simulink model "ieee30"  (R2017a)
settings: Solver=VariableStepDiscrete  StartTime=0.0  StopTime=0.012  MaxStep=1e-4  RelTol=1e-3
undefined symbols (not defined in the file): Angle, Magnitude
libraries: powerlib x548
(part 1 of 4)
settings Model: Creator=wynston  LastModifiedBy=Wynston
settings DataIOCC: ReturnWorkspaceOutputsName=simout

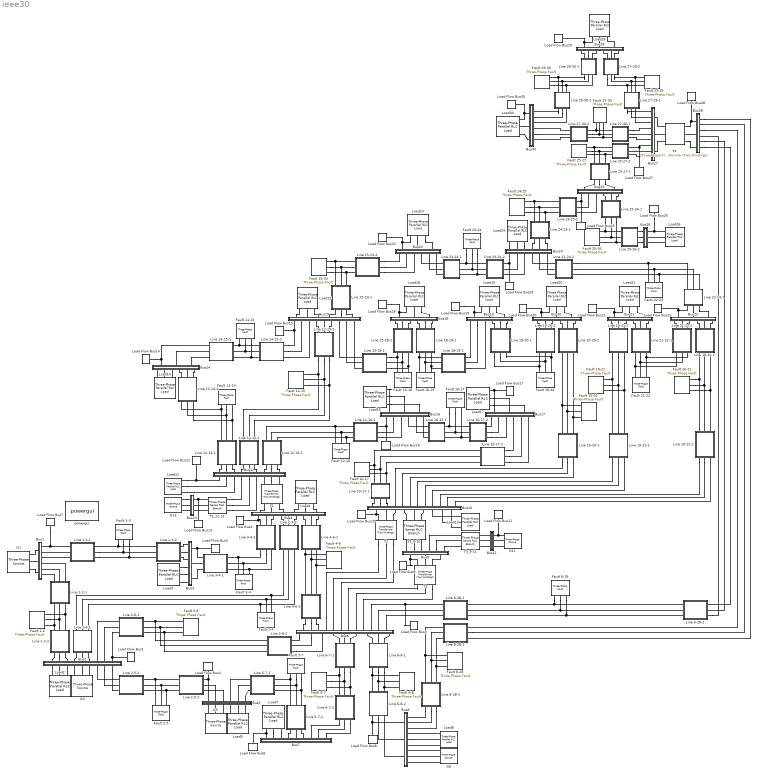
== system ieee30 ==
  Bus1 : Subsystem
  Bus10 : Subsystem
  Bus11 : Subsystem
  Bus12 : Subsystem
  Bus13 : Subsystem
  Bus14 : Subsystem
  Bus15 : Subsystem
  Bus16 : Subsystem
  Bus17 : Subsystem
  Bus18 : Subsystem
  Bus19 : Subsystem
  Bus2 : Subsystem
  Bus20 : Subsystem
  Bus21 : Subsystem
  Bus22 : Subsystem
  Bus23 : Subsystem
  Bus24 : Subsystem
  Bus25 : Subsystem
  Bus26 : Subsystem
  Bus27 : Subsystem
  Bus28 : Subsystem
  Bus29 : Subsystem
  Bus3 : Subsystem
  Bus30 : Subsystem
  Bus4 : Subsystem
  Bus5 : Subsystem
  Bus6 : Subsystem
  Bus7 : Subsystem
  Bus8 : Subsystem
  Bus9 : Subsystem
  Fault 1-2 : powerlib/Elements/Three-Phase Fault  InitialStates=0  FaultA=off  FaultB=off  FaultC=off  GroundFault=off  SwitchTimes=[0.008 0.1]  External=off  SwitchStatus=NaN  FaultResistance=0.001  GroundResistance=0.001  SnubberResistance=1e6  SnubberCapacitance=inf  Measurements=None
  Fault 1-3 : powerlib/Elements/Three-Phase Fault  InitialStates=0  FaultA=off  FaultB=off  FaultC=off  GroundFault=off  SwitchTimes=[0.008 0.1]  External=off  SwitchStatus=NaN  FaultResistance=0.001  GroundResistance=0.001  SnubberResistance=1e6  SnubberCapacitance=inf  Measurements=None
  Fault 10-{17,20..22} (4 alike) : powerlib/Elements/Three-Phase Fault  InitialStates=0  FaultA=off  FaultB=off  FaultC=off  GroundFault=off  SwitchTimes=[0.008 0.1]  External=off  SwitchStatus=NaN  FaultResistance=0.001  GroundResistance=0.001  SnubberResistance=1e6  SnubberCapacitance=inf  Measurements=None
  Fault 12-14 : powerlib/Elements/Three-Phase Fault  InitialStates=0  FaultA=off  FaultB=off  FaultC=off  GroundFault=off  SwitchTimes=[0.008 0.1]  External=off  SwitchStatus=NaN  FaultResistance=0.001  GroundResistance=0.001  SnubberResistance=1e6  SnubberCapacitance=inf  Measurements=None
  Fault 12-15 : powerlib/Elements/Three-Phase Fault  InitialStates=0  FaultA=off  FaultB=off  FaultC=off  GroundFault=off  SwitchTimes=[0.008 0.1]  External=off  SwitchStatus=NaN  FaultResistance=0.001  GroundResistance=0.001  SnubberResistance=1e6  SnubberCapacitance=inf  Measurements=None
  Fault 12-16 : powerlib/Elements/Three-Phase Fault  InitialStates=0  FaultA=off  FaultB=off  FaultC=off  GroundFault=off  SwitchTimes=[0.008 0.1]  External=off  SwitchStatus=NaN  FaultResistance=0.001  GroundResistance=0.001  SnubberResistance=1e6  SnubberCapacitance=inf  Measurements=None
  Fault 14-15 : powerlib/Elements/Three-Phase Fault  InitialStates=0  FaultA=off  FaultB=off  FaultC=off  GroundFault=off  SwitchTimes=[0.008 0.1]  External=off  SwitchStatus=NaN  FaultResistance=0.001  GroundResistance=0.001  SnubberResistance=1e6  SnubberCapacitance=inf  Measurements=None
  Fault 15-18 : powerlib/Elements/Three-Phase Fault  InitialStates=0  FaultA=off  FaultB=off  FaultC=off  GroundFault=off  SwitchTimes=[0.008 0.1]  External=off  SwitchStatus=NaN  FaultResistance=0.001  GroundResistance=0.001  SnubberResistance=1e6  SnubberCapacitance=inf  Measurements=None
  Fault 15-23 : powerlib/Elements/Three-Phase Fault  InitialStates=0  FaultA=off  FaultB=off  FaultC=off  GroundFault=off  SwitchTimes=[0.008 0.1]  External=off  SwitchStatus=NaN  FaultResistance=0.001  GroundResistance=0.001  SnubberResistance=1e6  SnubberCapacitance=inf  Measurements=None
  Fault 16-17 : powerlib/Elements/Three-Phase Fault  InitialStates=0  FaultA=off  FaultB=off  FaultC=off  GroundFault=off  SwitchTimes=[0.008 0.1]  External=off  SwitchStatus=NaN  FaultResistance=0.001  GroundResistance=0.001  SnubberResistance=1e6  SnubberCapacitance=inf  Measurements=None
  Fault 18-19 : powerlib/Elements/Three-Phase Fault  InitialStates=0  FaultA=off  FaultB=off  FaultC=off  GroundFault=off  SwitchTimes=[0.008 0.1]  External=off  SwitchStatus=NaN  FaultResistance=0.001  GroundResistance=0.001  SnubberResistance=1e6  SnubberCapacitance=inf  Measurements=None
  Fault 19-20 : powerlib/Elements/Three-Phase Fault  InitialStates=0  FaultA=off  FaultB=off  FaultC=off  GroundFault=off  SwitchTimes=[0.008 0.1]  External=off  SwitchStatus=NaN  FaultResistance=0.001  GroundResistance=0.001  SnubberResistance=1e6  SnubberCapacitance=inf  Measurements=None
  Fault 2-4 : powerlib/Elements/Three-Phase Fault  InitialStates=0  FaultA=off  FaultB=off  FaultC=off  GroundFault=off  SwitchTimes=[0.008 0.1]  External=off  SwitchStatus=NaN  FaultResistance=0.001  GroundResistance=0.001  SnubberResistance=1e6  SnubberCapacitance=inf  Measurements=None
  Fault 2-5 : powerlib/Elements/Three-Phase Fault  InitialStates=0  FaultA=off  FaultB=off  FaultC=off  GroundFault=off  SwitchTimes=[0.008 0.1]  External=off  SwitchStatus=NaN  FaultResistance=0.001  GroundResistance=0.001  SnubberResistance=1e6  SnubberCapacitance=inf  Measurements=None
  Fault 2-6 : powerlib/Elements/Three-Phase Fault  InitialStates=0  FaultA=off  FaultB=off  FaultC=off  GroundFault=off  SwitchTimes=[0.008 0.1]  External=off  SwitchStatus=NaN  FaultResistance=0.001  GroundResistance=0.001  SnubberResistance=1e6  SnubberCapacitance=inf  Measurements=None
  Fault 21-22 : powerlib/Elements/Three-Phase Fault  InitialStates=0  FaultA=off  FaultB=off  FaultC=off  GroundFault=off  SwitchTimes=[0.008 0.1]  External=off  SwitchStatus=NaN  FaultResistance=0.001  GroundResistance=0.001  SnubberResistance=1e6  SnubberCapacitance=inf  Measurements=None
  Fault 22-24 : powerlib/Elements/Three-Phase Fault  InitialStates=0  FaultA=off  FaultB=off  FaultC=off  GroundFault=off  SwitchTimes=[0.008 0.1]  External=off  SwitchStatus=NaN  FaultResistance=0.001  GroundResistance=0.001  SnubberResistance=1e6  SnubberCapacitance=inf  Measurements=None
  Fault 23-24 : powerlib/Elements/Three-Phase Fault  InitialStates=0  FaultA=off  FaultB=off  FaultC=off  GroundFault=off  SwitchTimes=[0.008 0.1]  External=off  SwitchStatus=NaN  FaultResistance=0.001  GroundResistance=0.001  SnubberResistance=1e6  SnubberCapacitance=inf  Measurements=None
  Fault 24-25 : powerlib/Elements/Three-Phase Fault  InitialStates=0  FaultA=off  FaultB=off  FaultC=off  GroundFault=off  SwitchTimes=[0.008 0.1]  External=off  SwitchStatus=NaN  FaultResistance=0.001  GroundResistance=0.001  SnubberResistance=1e6  SnubberCapacitance=inf  Measurements=None
  Fault 25-26 : powerlib/Elements/Three-Phase Fault  InitialStates=0  FaultA=off  FaultB=off  FaultC=off  GroundFault=off  SwitchTimes=[0.008 0.1]  External=off  SwitchStatus=NaN  FaultResistance=0.001  GroundResistance=0.001  SnubberResistance=1e6  SnubberCapacitance=inf  Measurements=None
  Fault 25-27 : powerlib/Elements/Three-Phase Fault  InitialStates=0  FaultA=off  FaultB=off  FaultC=off  GroundFault=off  SwitchTimes=[0.008 0.1]  External=off  SwitchStatus=NaN  FaultResistance=0.001  GroundResistance=0.001  SnubberResistance=1e6  SnubberCapacitance=inf  Measurements=None
  Fault 27-29 : powerlib/Elements/Three-Phase Fault  InitialStates=0  FaultA=off  FaultB=off  FaultC=off  GroundFault=off  SwitchTimes=[0.008 0.1]  External=off  SwitchStatus=NaN  FaultResistance=0.001  GroundResistance=0.001  SnubberResistance=1e6  SnubberCapacitance=inf  Measurements=None
  Fault 27-30 : powerlib/Elements/Three-Phase Fault  InitialStates=0  FaultA=off  FaultB=off  FaultC=off  GroundFault=off  SwitchTimes=[0.008 0.1]  External=off  SwitchStatus=NaN  FaultResistance=0.001  GroundResistance=0.001  SnubberResistance=1e6  SnubberCapacitance=inf  Measurements=None
  Fault 29-30 : powerlib/Elements/Three-Phase Fault  InitialStates=0  FaultA=off  FaultB=off  FaultC=off  GroundFault=off  SwitchTimes=[0.008 0.1]  External=off  SwitchStatus=NaN  FaultResistance=0.001  GroundResistance=0.001  SnubberResistance=1e6  SnubberCapacitance=inf  Measurements=None
  Fault 3-4 : powerlib/Elements/Three-Phase Fault  InitialStates=0  FaultA=off  FaultB=off  FaultC=off  GroundFault=off  SwitchTimes=[0.008 0.1]  External=off  SwitchStatus=NaN  FaultResistance=0.001  GroundResistance=0.001  SnubberResistance=1e6  SnubberCapacitance=inf  Measurements=None
  Fault 4-6 : powerlib/Elements/Three-Phase Fault  InitialStates=0  FaultA=off  FaultB=off  FaultC=off  GroundFault=off  SwitchTimes=[0.008 0.1]  External=off  SwitchStatus=NaN  FaultResistance=0.001  GroundResistance=0.001  SnubberResistance=1e6  SnubberCapacitance=inf  Measurements=None
  Fault 5-7 : powerlib/Elements/Three-Phase Fault  InitialStates=0  FaultA=off  FaultB=off  FaultC=off  GroundFault=off  SwitchTimes=[0.008 0.1]  External=off  SwitchStatus=NaN  FaultResistance=0.001  GroundResistance=0.001  SnubberResistance=1e6  SnubberCapacitance=inf  Measurements=None
  Fault 6-28 : powerlib/Elements/Three-Phase Fault  InitialStates=0  FaultA=off  FaultB=off  FaultC=off  GroundFault=off  SwitchTimes=[0.008 0.1]  External=off  SwitchStatus=NaN  FaultResistance=0.001  GroundResistance=0.001  SnubberResistance=1e6  SnubberCapacitance=inf  Measurements=None
  Fault 6-7 : powerlib/Elements/Three-Phase Fault  InitialStates=0  FaultA=off  FaultB=off  FaultC=off  GroundFault=off  SwitchTimes=[0.008 0.1]  External=off  SwitchStatus=NaN  FaultResistance=0.001  GroundResistance=0.001  SnubberResistance=1e6  SnubberCapacitance=inf  Measurements=None
  Fault 6-8 : powerlib/Elements/Three-Phase Fault  InitialStates=0  FaultA=off  FaultB=off  FaultC=off  GroundFault=off  SwitchTimes=[0.008 0.1]  External=off  SwitchStatus=NaN  FaultResistance=0.001  GroundResistance=0.001  SnubberResistance=1e6  SnubberCapacitance=inf  Measurements=None
  Fault 8-28 : powerlib/Elements/Three-Phase Fault  InitialStates=0  FaultA=off  FaultB=off  FaultC=off  GroundFault=off  SwitchTimes=[0.008 0.1]  External=off  SwitchStatus=NaN  FaultResistance=0.001  GroundResistance=0.001  SnubberResistance=1e6  SnubberCapacitance=inf  Measurements=None
  G1 : powerlib/Electrical Sources/Three-Phase Source  InternalConnection=Yg  VoltagePhases=off  Voltage=(132000)*2.93771  PhaseAngle=58.3306  Voltage_phases=[25e3 25e3 25e3]/sqrt(3)  PhaseAngles_phases=[0 -120 +120]  Frequency=60  NonIdealSource=on  SpecifyImpedance=on  Resistance=0.8929  Inductance=16.58e-3  ShortCircuitLevel=100e6  BaseVoltage=132e3  XRratio=100000  BusType=swing  Pref=0e6  Qref=0  Prefabc=[10e3, 10e3, 10e3]  Qrefabc=[0, 0, 0]  Qmin=0e6  Qmax=0e6
  G11 : powerlib/Electrical Sources/Three-Phase Source  InternalConnection=Yg  VoltagePhases=off  Voltage=(33000)*1.10022  PhaseAngle=-11.1711  Voltage_phases=[25e3 25e3 25e3]/sqrt(3)  PhaseAngles_phases=[0 -120 +120]  Frequency=60  NonIdealSource=on  SpecifyImpedance=on  Resistance=0.8929  Inductance=16.58e-3  ShortCircuitLevel=100e6  BaseVoltage=33e3  XRratio=100000  BusType=PV  Pref=0e6  Qref=0  Prefabc=[10e3, 10e3, 10e3]  Qrefabc=[0, 0, 0]  Qmin=-6e6  Qmax=24e6
  G13 : powerlib/Electrical Sources/Three-Phase Source  InternalConnection=Yg  VoltagePhases=off  Voltage=(33000)*1.10798  PhaseAngle=-18.3402  Voltage_phases=[25e3 25e3 25e3]/sqrt(3)  PhaseAngles_phases=[0 -120 +120]  Frequency=60  NonIdealSource=on  SpecifyImpedance=on  Resistance=0.8929  Inductance=16.58e-3  ShortCircuitLevel=100e6  BaseVoltage=32e3  XRratio=100000  BusType=PV  Pref=0e6  Qref=0  Prefabc=[10e3, 10e3, 10e3]  Qrefabc=[0, 0, 0]  Qmin=-6e6  Qmax=24e6
  G2 : powerlib/Electrical Sources/Three-Phase Source  InternalConnection=Yg  VoltagePhases=off  Voltage=(132000)*1.55993  PhaseAngle=9.4414  Voltage_phases=[25e3 25e3 25e3]/sqrt(3)  PhaseAngles_phases=[0 -120 +120]  Frequency=60  NonIdealSource=on  SpecifyImpedance=on  Resistance=0.8929  Inductance=16.58e-3  ShortCircuitLevel=100e6  BaseVoltage=132e3  XRratio=100000  BusType=PV  Pref=40e6  Qref=0  Prefabc=[10e3, 10e3, 10e3]  Qrefabc=[0, 0, 0]  Qmin=-40e6  Qmax=50e6
  G5 : powerlib/Electrical Sources/Three-Phase Source  InternalConnection=Yg  VoltagePhases=off  Voltage=(132000)*1.38256  PhaseAngle=-14.4167  Voltage_phases=[25e3 25e3 25e3]/sqrt(3)  PhaseAngles_phases=[0 -120 +120]  Frequency=60  NonIdealSource=on  SpecifyImpedance=on  Resistance=0.8929  Inductance=16.58e-3  ShortCircuitLevel=100e6  BaseVoltage=132e3  XRratio=100000  BusType=PV  Pref=0e6  Qref=0  Prefabc=[10e3, 10e3, 10e3]  Qrefabc=[0, 0, 0]  Qmin=-40e6  Qmax=40e6
  G8 : powerlib/Electrical Sources/Three-Phase Source  InternalConnection=Yg  VoltagePhases=off  Voltage=(132000)*1.37308  PhaseAngle=-11.5895  Voltage_phases=[25e3 25e3 25e3]/sqrt(3)  PhaseAngles_phases=[0 -120 +120]  Frequency=60  NonIdealSource=on  SpecifyImpedance=on  Resistance=0.8929  Inductance=16.58e-3  ShortCircuitLevel=100e6  BaseVoltage=132e3  XRratio=100000  BusType=PV  Pref=0e6  Qref=0  Prefabc=[10e3, 10e3, 10e3]  Qrefabc=[0, 0, 0]  Qmin=-10e6  Qmax=40e6
  Line 1-2-1 : Subsystem  mask{R=0.0096, X=0.02875, B=0.0132, MVA=100, KV=132}
      mask prompts: R "Resistance (pu)"; X "Reactance(pu)"; B "Susceptance (pu)(B/2)"; MVA "MVA Base"; KV "KV Base"
      mask help: Transmission Line Pi model
      mask init:
      | rt = R*(KV^2)/MVA;
      | lt = (X/377)*(KV^2)/MVA;
      | ct = (2*B/377)/((KV^2)/MVA);
      | ro = 2.5*R*(KV^2)/MVA;
      | lo = 2.5*(X/377)*(KV^2)/MVA;
      | co = (2*B/377)/((1.6*KV^2)/MVA);
      mask Display:
      | plot([0.2 0.8 0.8 0.2 0.2], [0.35 0.35 0.65 0.65 0.35]);
      | text(0.5, 0.5, 'π', 'horizontalAlignment', 'center');
  Line 1-2-2 : Subsystem  mask{R=0.0096, X=0.02875, B=0.0132, MVA=100, KV=132}
      mask prompts: R "Resistance (pu)"; X "Reactance(pu)"; B "Susceptance (pu)(B/2)"; MVA "MVA Base"; KV "KV Base"
      mask help: Transmission Line Pi model
      mask init:
      | rt = R*(KV^2)/MVA;
      | lt = (X/377)*(KV^2)/MVA;
      | ct = (2*B/377)/((KV^2)/MVA);
      | ro = 2.5*R*(KV^2)/MVA;
      | lo = 2.5*(X/377)*(KV^2)/MVA;
      | co = (2*B/377)/((1.6*KV^2)/MVA);
      mask Display:
      | plot([0.2 0.8 0.8 0.2 0.2], [0.35 0.35 0.65 0.65 0.35]);
      | text(0.5, 0.5, 'π', 'horizontalAlignment', 'center');
  Line 1-3-1 : Subsystem  mask{R=0.0226, X=0.0825, B=0.0102, MVA=100, KV=132}
      mask prompts: R "Resistance (pu)"; X "Reactance(pu)"; B "Susceptance (pu)(B/2)"; MVA "MVA Base"; KV "KV Base"
      mask help: Transmission Line Pi model
      mask init:
      | rt = R*(KV^2)/MVA;
      | lt = (X/377)*(KV^2)/MVA;
      | ct = (2*B/377)/((KV^2)/MVA);
      | ro = 2.5*R*(KV^2)/MVA;
      | lo = 2.5*(X/377)*(KV^2)/MVA;
      | co = (2*B/377)/((1.6*KV^2)/MVA);
      mask Display:
      | plot([0.2 0.8 0.8 0.2 0.2], [0.35 0.35 0.65 0.65 0.35]);
      | text(0.5, 0.5, 'π', 'horizontalAlignment', 'center');
  Line 1-3-2 : Subsystem  mask{R=0.0226, X=0.0825, B=0.0102, MVA=100, KV=132}
      mask prompts: R "Resistance (pu)"; X "Reactance(pu)"; B "Susceptance (pu)(B/2)"; MVA "MVA Base"; KV "KV Base"
      mask help: Transmission Line Pi model
      mask init:
      | rt = R*(KV^2)/MVA;
      | lt = (X/377)*(KV^2)/MVA;
      | ct = (2*B/377)/((KV^2)/MVA);
      | ro = 2.5*R*(KV^2)/MVA;
      | lo = 2.5*(X/377)*(KV^2)/MVA;
      | co = (2*B/377)/((1.6*KV^2)/MVA);
      mask Display:
      | plot([0.2 0.8 0.8 0.2 0.2], [0.35 0.35 0.65 0.65 0.35]);
      | text(0.5, 0.5, 'π', 'horizontalAlignment', 'center');
  Line 10-17-1 : Subsystem  mask{R=0.0162, X=0.04225, B=2.5e-05, MVA=100, KV=33}
      mask prompts: R "Resistance (pu)"; X "Reactance(pu)"; B "Susceptance (pu)(B/2)"; MVA "MVA Base"; KV "KV Base"
      mask help: Transmission Line Pi model
      mask init:
      | rt = R*(KV^2)/MVA;
      | lt = (X/377)*(KV^2)/MVA;
      | ct = (2*B/377)/((KV^2)/MVA);
      | ro = 2.5*R*(KV^2)/MVA;
      | lo = 2.5*(X/377)*(KV^2)/MVA;
      | co = (2*B/377)/((1.6*KV^2)/MVA);
      mask Display:
      | plot([0.2 0.8 0.8 0.2 0.2], [0.35 0.35 0.65 0.65 0.35]);
      | text(0.5, 0.5, 'π', 'horizontalAlignment', 'center');
  Line 10-17-2 : Subsystem  mask{R=0.0162, X=0.04225, B=2.5e-05, MVA=100, KV=33}
      mask prompts: R "Resistance (pu)"; X "Reactance(pu)"; B "Susceptance (pu)(B/2)"; MVA "MVA Base"; KV "KV Base"
      mask help: Transmission Line Pi model
      mask init:
      | rt = R*(KV^2)/MVA;
      | lt = (X/377)*(KV^2)/MVA;
      | ct = (2*B/377)/((KV^2)/MVA);
      | ro = 2.5*R*(KV^2)/MVA;
      | lo = 2.5*(X/377)*(KV^2)/MVA;
      | co = (2*B/377)/((1.6*KV^2)/MVA);
      mask Display:
      | plot([0.2 0.8 0.8 0.2 0.2], [0.35 0.35 0.65 0.65 0.35]);
      | text(0.5, 0.5, 'π', 'horizontalAlignment', 'center');
  Line 10-20-1 : Subsystem  mask{R=0.0468, X=0.1045, B=2.5e-05, MVA=100, KV=33}
      mask prompts: R "Resistance (pu)"; X "Reactance(pu)"; B "Susceptance (pu)(B/2)"; MVA "MVA Base"; KV "KV Base"
      mask help: Transmission Line Pi model
      mask init:
      | rt = R*(KV^2)/MVA;
      | lt = (X/377)*(KV^2)/MVA;
      | ct = (2*B/377)/((KV^2)/MVA);
      | ro = 2.5*R*(KV^2)/MVA;
      | lo = 2.5*(X/377)*(KV^2)/MVA;
      | co = (2*B/377)/((1.6*KV^2)/MVA);
      mask Display:
      | plot([0.2 0.8 0.8 0.2 0.2], [0.35 0.35 0.65 0.65 0.35]);
      | text(0.5, 0.5, 'π', 'horizontalAlignment', 'center');
  Line 10-20-2 : Subsystem  mask{R=0.0468, X=0.1045, B=2.5e-05, MVA=100, KV=33}
      mask prompts: R "Resistance (pu)"; X "Reactance(pu)"; B "Susceptance (pu)(B/2)"; MVA "MVA Base"; KV "KV Base"
      mask help: Transmission Line Pi model
      mask init:
      | rt = R*(KV^2)/MVA;
      | lt = (X/377)*(KV^2)/MVA;
      | ct = (2*B/377)/((KV^2)/MVA);
      | ro = 2.5*R*(KV^2)/MVA;
      | lo = 2.5*(X/377)*(KV^2)/MVA;
      | co = (2*B/377)/((1.6*KV^2)/MVA);
      mask Display:
      | plot([0.2 0.8 0.8 0.2 0.2], [0.35 0.35 0.65 0.65 0.35]);
      | text(0.5, 0.5, 'π', 'horizontalAlignment', 'center');
  Line 10-21-1 : Subsystem  mask{R=0.0174, X=0.03745, B=2.5e-05, MVA=100, KV=33}
      mask prompts: R "Resistance (pu)"; X "Reactance(pu)"; B "Susceptance (pu)(B/2)"; MVA "MVA Base"; KV "KV Base"
      mask help: Transmission Line Pi model
      mask init:
      | rt = R*(KV^2)/MVA;
      | lt = (X/377)*(KV^2)/MVA;
      | ct = (2*B/377)/((KV^2)/MVA);
      | ro = 2.5*R*(KV^2)/MVA;
      | lo = 2.5*(X/377)*(KV^2)/MVA;
      | co = (2*B/377)/((1.6*KV^2)/MVA);
      mask Display:
      | plot([0.2 0.8 0.8 0.2 0.2], [0.35 0.35 0.65 0.65 0.35]);
      | text(0.5, 0.5, 'π', 'horizontalAlignment', 'center');
  Line 10-21-2 : Subsystem  mask{R=0.0174, X=0.03745, B=2.5e-05, MVA=100, KV=33}
      mask prompts: R "Resistance (pu)"; X "Reactance(pu)"; B "Susceptance (pu)(B/2)"; MVA "MVA Base"; KV "KV Base"
      mask help: Transmission Line Pi model
      mask init:
      | rt = R*(KV^2)/MVA;
      | lt = (X/377)*(KV^2)/MVA;
      | ct = (2*B/377)/((KV^2)/MVA);
      | ro = 2.5*R*(KV^2)/MVA;
      | lo = 2.5*(X/377)*(KV^2)/MVA;
      | co = (2*B/377)/((1.6*KV^2)/MVA);
      mask Display:
      | plot([0.2 0.8 0.8 0.2 0.2], [0.35 0.35 0.65 0.65 0.35]);
      | text(0.5, 0.5, 'π', 'horizontalAlignment', 'center');
  Line 10-22-1 : Subsystem  mask{R=0.03635, X=0.075, B=2.5e-05, MVA=100, KV=33}
      mask prompts: R "Resistance (pu)"; X "Reactance(pu)"; B "Susceptance (pu)(B/2)"; MVA "MVA Base"; KV "KV Base"
      mask help: Transmission Line Pi model
      mask init:
      | rt = R*(KV^2)/MVA;
      | lt = (X/377)*(KV^2)/MVA;
      | ct = (2*B/377)/((KV^2)/MVA);
      | ro = 2.5*R*(KV^2)/MVA;
      | lo = 2.5*(X/377)*(KV^2)/MVA;
      | co = (2*B/377)/((1.6*KV^2)/MVA);
      mask Display:
      | plot([0.2 0.8 0.8 0.2 0.2], [0.35 0.35 0.65 0.65 0.35]);
      | text(0.5, 0.5, 'π', 'horizontalAlignment', 'center');
  Line 10-22-2 : Subsystem  mask{R=0.03635, X=0.075, B=2.5e-05, MVA=100, KV=33}
      mask prompts: R "Resistance (pu)"; X "Reactance(pu)"; B "Susceptance (pu)(B/2)"; MVA "MVA Base"; KV "KV Base"
      mask help: Transmission Line Pi model
      mask init:
      | rt = R*(KV^2)/MVA;
      | lt = (X/377)*(KV^2)/MVA;
      | ct = (2*B/377)/((KV^2)/MVA);
      | ro = 2.5*R*(KV^2)/MVA;
      | lo = 2.5*(X/377)*(KV^2)/MVA;
      | co = (2*B/377)/((1.6*KV^2)/MVA);
      mask Display:
      | plot([0.2 0.8 0.8 0.2 0.2], [0.35 0.35 0.65 0.65 0.35]);
      | text(0.5, 0.5, 'π', 'horizontalAlignment', 'center');
  Line 12-14-1 : Subsystem  mask{R=0.0615, X=0.128, B=2.5e-05, MVA=100, KV=33}
      mask prompts: R "Resistance (pu)"; X "Reactance(pu)"; B "Susceptance (pu)(B/2)"; MVA "MVA Base"; KV "KV Base"
      mask help: Transmission Line Pi model
      mask init:
      | rt = R*(KV^2)/MVA;
      | lt = (X/377)*(KV^2)/MVA;
      | ct = (2*B/377)/((KV^2)/MVA);
      | ro = 2.5*R*(KV^2)/MVA;
      | lo = 2.5*(X/377)*(KV^2)/MVA;
      | co = (2*B/377)/((1.6*KV^2)/MVA);
      mask Display:
      | plot([0.2 0.8 0.8 0.2 0.2], [0.35 0.35 0.65 0.65 0.35]);
      | text(0.5, 0.5, 'π', 'horizontalAlignment', 'center');
  Line 12-14-2 : Subsystem  mask{R=0.0615, X=0.128, B=2.5e-05, MVA=100, KV=33}
      mask prompts: R "Resistance (pu)"; X "Reactance(pu)"; B "Susceptance (pu)(B/2)"; MVA "MVA Base"; KV "KV Base"
      mask help: Transmission Line Pi model
      mask init:
      | rt = R*(KV^2)/MVA;
      | lt = (X/377)*(KV^2)/MVA;
      | ct = (2*B/377)/((KV^2)/MVA);
      | ro = 2.5*R*(KV^2)/MVA;
      | lo = 2.5*(X/377)*(KV^2)/MVA;
      | co = (2*B/377)/((1.6*KV^2)/MVA);
      mask Display:
      | plot([0.2 0.8 0.8 0.2 0.2], [0.35 0.35 0.65 0.65 0.35]);
      | text(0.5, 0.5, 'π', 'horizontalAlignment', 'center');
  Line 12-15-1 : Subsystem  mask{R=0.0331, X=0.065, B=2.5e-05, MVA=100, KV=33}
      mask prompts: R "Resistance (pu)"; X "Reactance(pu)"; B "Susceptance (pu)(B/2)"; MVA "MVA Base"; KV "KV Base"
      mask help: Transmission Line Pi model
      mask init:
      | rt = R*(KV^2)/MVA;
      | lt = (X/377)*(KV^2)/MVA;
      | ct = (2*B/377)/((KV^2)/MVA);
      | ro = 2.5*R*(KV^2)/MVA;
      | lo = 2.5*(X/377)*(KV^2)/MVA;
      | co = (2*B/377)/((1.6*KV^2)/MVA);
      mask Display:
      | plot([0.2 0.8 0.8 0.2 0.2], [0.35 0.35 0.65 0.65 0.35]);
      | text(0.5, 0.5, 'π', 'horizontalAlignment', 'center');
  Line 12-15-2 : Subsystem  mask{R=0.0331, X=0.065, B=2.5e-05, MVA=100, KV=33}
      mask prompts: R "Resistance (pu)"; X "Reactance(pu)"; B "Susceptance (pu)(B/2)"; MVA "MVA Base"; KV "KV Base"
      mask help: Transmission Line Pi model
      mask init:
      | rt = R*(KV^2)/MVA;
      | lt = (X/377)*(KV^2)/MVA;
      | ct = (2*B/377)/((KV^2)/MVA);
      | ro = 2.5*R*(KV^2)/MVA;
      | lo = 2.5*(X/377)*(KV^2)/MVA;
      | co = (2*B/377)/((1.6*KV^2)/MVA);
      mask Display:
      | plot([0.2 0.8 0.8 0.2 0.2], [0.35 0.35 0.65 0.65 0.35]);
      | text(0.5, 0.5, 'π', 'horizontalAlignment', 'center');
  Line 12-16-1 : Subsystem  mask{R=0.04725, X=0.0995, B=2.5e-05, MVA=100, KV=33}
      mask prompts: R "Resistance (pu)"; X "Reactance(pu)"; B "Susceptance (pu)(B/2)"; MVA "MVA Base"; KV "KV Base"
      mask help: Transmission Line Pi model
      mask init:
      | rt = R*(KV^2)/MVA;
      | lt = (X/377)*(KV^2)/MVA;
      | ct = (2*B/377)/((KV^2)/MVA);
      | ro = 2.5*R*(KV^2)/MVA;
      | lo = 2.5*(X/377)*(KV^2)/MVA;
      | co = (2*B/377)/((1.6*KV^2)/MVA);
      mask Display:
      | plot([0.2 0.8 0.8 0.2 0.2], [0.35 0.35 0.65 0.65 0.35]);
      | text(0.5, 0.5, 'π', 'horizontalAlignment', 'center');
  Line 12-16-2 : Subsystem  mask{R=0.04725, X=0.0995, B=2.5e-05, MVA=100, KV=33}
      mask prompts: R "Resistance (pu)"; X "Reactance(pu)"; B "Susceptance (pu)(B/2)"; MVA "MVA Base"; KV "KV Base"
      mask help: Transmission Line Pi model
      mask init:
      | rt = R*(KV^2)/MVA;
      | lt = (X/377)*(KV^2)/MVA;
      | ct = (2*B/377)/((KV^2)/MVA);
      | ro = 2.5*R*(KV^2)/MVA;
      | lo = 2.5*(X/377)*(KV^2)/MVA;
      | co = (2*B/377)/((1.6*KV^2)/MVA);
      mask Display:
      | plot([0.2 0.8 0.8 0.2 0.2], [0.35 0.35 0.65 0.65 0.35]);
      | text(0.5, 0.5, 'π', 'horizontalAlignment', 'center');
  Line 14-15-1 : Subsystem  mask{R=0.1105, X=0.1, B=2.5e-05, MVA=100, KV=33}
      mask prompts: R "Resistance (pu)"; X "Reactance(pu)"; B "Susceptance (pu)(B/2)"; MVA "MVA Base"; KV "KV Base"
      mask help: Transmission Line Pi model
      mask init:
      | rt = R*(KV^2)/MVA;
      | lt = (X/377)*(KV^2)/MVA;
      | ct = (2*B/377)/((KV^2)/MVA);
      | ro = 2.5*R*(KV^2)/MVA;
      | lo = 2.5*(X/377)*(KV^2)/MVA;
      | co = (2*B/377)/((1.6*KV^2)/MVA);
      mask Display:
      | plot([0.2 0.8 0.8 0.2 0.2], [0.35 0.35 0.65 0.65 0.35]);
      | text(0.5, 0.5, 'π', 'horizontalAlignment', 'center');
  Line 14-15-2 : Subsystem  mask{R=0.1105, X=0.1, B=2.5e-05, MVA=100, KV=33}
      mask prompts: R "Resistance (pu)"; X "Reactance(pu)"; B "Susceptance (pu)(B/2)"; MVA "MVA Base"; KV "KV Base"
      mask help: Transmission Line Pi model
      mask init:
      | rt = R*(KV^2)/MVA;
      | lt = (X/377)*(KV^2)/MVA;
      | ct = (2*B/377)/((KV^2)/MVA);
      | ro = 2.5*R*(KV^2)/MVA;
      | lo = 2.5*(X/377)*(KV^2)/MVA;
      | co = (2*B/377)/((1.6*KV^2)/MVA);
      mask Display:
      | plot([0.2 0.8 0.8 0.2 0.2], [0.35 0.35 0.65 0.65 0.35]);
      | text(0.5, 0.5, 'π', 'horizontalAlignment', 'center');
  Line 15-18-1 : Subsystem  mask{R=0.0535, X=0.1095, B=2.5e-05, MVA=100, KV=33}
      mask prompts: R "Resistance (pu)"; X "Reactance(pu)"; B "Susceptance (pu)(B/2)"; MVA "MVA Base"; KV "KV Base"
      mask help: Transmission Line Pi model
      mask init:
      | rt = R*(KV^2)/MVA;
      | lt = (X/377)*(KV^2)/MVA;
      | ct = (2*B/377)/((KV^2)/MVA);
      | ro = 2.5*R*(KV^2)/MVA;
      | lo = 2.5*(X/377)*(KV^2)/MVA;
      | co = (2*B/377)/((1.6*KV^2)/MVA);
      mask Display:
      | plot([0.2 0.8 0.8 0.2 0.2], [0.35 0.35 0.65 0.65 0.35]);
      | text(0.5, 0.5, 'π', 'horizontalAlignment', 'center');
  Line 15-18-2 : Subsystem  mask{R=0.0535, X=0.1095, B=2.5e-05, MVA=100, KV=33}
      mask prompts: R "Resistance (pu)"; X "Reactance(pu)"; B "Susceptance (pu)(B/2)"; MVA "MVA Base"; KV "KV Base"
      mask help: Transmission Line Pi model
      mask init:
      | rt = R*(KV^2)/MVA;
      | lt = (X/377)*(KV^2)/MVA;
      | ct = (2*B/377)/((KV^2)/MVA);
      | ro = 2.5*R*(KV^2)/MVA;
      | lo = 2.5*(X/377)*(KV^2)/MVA;
      | co = (2*B/377)/((1.6*KV^2)/MVA);
      mask Display:
      | plot([0.2 0.8 0.8 0.2 0.2], [0.35 0.35 0.65 0.65 0.35]);
      | text(0.5, 0.5, 'π', 'horizontalAlignment', 'center');
  Line 15-23-1 : Subsystem  mask{R=0.05, X=0.101, B=2.5e-05, MVA=100, KV=33}
      mask prompts: R "Resistance (pu)"; X "Reactance(pu)"; B "Susceptance (pu)(B/2)"; MVA "MVA Base"; KV "KV Base"
      mask help: Transmission Line Pi model
      mask init:
      | rt = R*(KV^2)/MVA;
      | lt = (X/377)*(KV^2)/MVA;
      | ct = (2*B/377)/((KV^2)/MVA);
      | ro = 2.5*R*(KV^2)/MVA;
      | lo = 2.5*(X/377)*(KV^2)/MVA;
      | co = (2*B/377)/((1.6*KV^2)/MVA);
      mask Display:
      | plot([0.2 0.8 0.8 0.2 0.2], [0.35 0.35 0.65 0.65 0.35]);
      | text(0.5, 0.5, 'π', 'horizontalAlignment', 'center');
  Line 15-23-2 : Subsystem  mask{R=0.05, X=0.101, B=2.5e-05, MVA=100, KV=33}
      mask prompts: R "Resistance (pu)"; X "Reactance(pu)"; B "Susceptance (pu)(B/2)"; MVA "MVA Base"; KV "KV Base"
      mask help: Transmission Line Pi model
      mask init:
      | rt = R*(KV^2)/MVA;
      | lt = (X/377)*(KV^2)/MVA;
      | ct = (2*B/377)/((KV^2)/MVA);
      | ro = 2.5*R*(KV^2)/MVA;
      | lo = 2.5*(X/377)*(KV^2)/MVA;
      | co = (2*B/377)/((1.6*KV^2)/MVA);
      mask Display:
      | plot([0.2 0.8 0.8 0.2 0.2], [0.35 0.35 0.65 0.65 0.35]);
      | text(0.5, 0.5, 'π', 'horizontalAlignment', 'center');
  Line 16-17-1 : Subsystem  mask{R=0.0262, X=0.096, B=2.5e-05, MVA=100, KV=33}
      mask prompts: R "Resistance (pu)"; X "Reactance(pu)"; B "Susceptance (pu)(B/2)"; MVA "MVA Base"; KV "KV Base"
      mask help: Transmission Line Pi model
      mask init:
      | rt = R*(KV^2)/MVA;
      | lt = (X/377)*(KV^2)/MVA;
      | ct = (2*B/377)/((KV^2)/MVA);
      | ro = 2.5*R*(KV^2)/MVA;
      | lo = 2.5*(X/377)*(KV^2)/MVA;
      | co = (2*B/377)/((1.6*KV^2)/MVA);
      mask Display:
      | plot([0.2 0.8 0.8 0.2 0.2], [0.35 0.35 0.65 0.65 0.35]);
      | text(0.5, 0.5, 'π', 'horizontalAlignment', 'center');
  Line 16-17-2 : Subsystem  mask{R=0.0262, X=0.096, B=2.5e-05, MVA=100, KV=33}
      mask prompts: R "Resistance (pu)"; X "Reactance(pu)"; B "Susceptance (pu)(B/2)"; MVA "MVA Base"; KV "KV Base"
      mask help: Transmission Line Pi model
      mask init:
      | rt = R*(KV^2)/MVA;
      | lt = (X/377)*(KV^2)/MVA;
      | ct = (2*B/377)/((KV^2)/MVA);
      | ro = 2.5*R*(KV^2)/MVA;
      | lo = 2.5*(X/377)*(KV^2)/MVA;
      | co = (2*B/377)/((1.6*KV^2)/MVA);
      mask Display:
      | plot([0.2 0.8 0.8 0.2 0.2], [0.35 0.35 0.65 0.65 0.35]);
      | text(0.5, 0.5, 'π', 'horizontalAlignment', 'center');
  Line 18-19-1 : Subsystem  mask{R=0.03195, X=0.0645, B=2.5e-05, MVA=100, KV=33}
      mask prompts: R "Resistance (pu)"; X "Reactance(pu)"; B "Susceptance (pu)(B/2)"; MVA "MVA Base"; KV "KV Base"
      mask help: Transmission Line Pi model
      mask init:
      | rt = R*(KV^2)/MVA;
      | lt = (X/377)*(KV^2)/MVA;
      | ct = (2*B/377)/((KV^2)/MVA);
      | ro = 2.5*R*(KV^2)/MVA;
      | lo = 2.5*(X/377)*(KV^2)/MVA;
      | co = (2*B/377)/((1.6*KV^2)/MVA);
      mask Display:
      | plot([0.2 0.8 0.8 0.2 0.2], [0.35 0.35 0.65 0.65 0.35]);
      | text(0.5, 0.5, 'π', 'horizontalAlignment', 'center');
  Line 18-19-2 : Subsystem  mask{R=0.03195, X=0.0645, B=2.5e-05, MVA=100, KV=33}
      mask prompts: R "Resistance (pu)"; X "Reactance(pu)"; B "Susceptance (pu)(B/2)"; MVA "MVA Base"; KV "KV Base"
      mask help: Transmission Line Pi model
      mask init:
      | rt = R*(KV^2)/MVA;
      | lt = (X/377)*(KV^2)/MVA;
      | ct = (2*B/377)/((KV^2)/MVA);
      | ro = 2.5*R*(KV^2)/MVA;
      | lo = 2.5*(X/377)*(KV^2)/MVA;
      | co = (2*B/377)/((1.6*KV^2)/MVA);
      mask Display:
      | plot([0.2 0.8 0.8 0.2 0.2], [0.35 0.35 0.65 0.65 0.35]);
      | text(0.5, 0.5, 'π', 'horizontalAlignment', 'center');
  Line 19-20-1 : Subsystem  mask{R=0.017, X=0.034, B=2.5e-05, MVA=100, KV=33}
      mask prompts: R "Resistance (pu)"; X "Reactance(pu)"; B "Susceptance (pu)(B/2)"; MVA "MVA Base"; KV "KV Base"
      mask help: Transmission Line Pi model
      mask init:
      | rt = R*(KV^2)/MVA;
      | lt = (X/377)*(KV^2)/MVA;
      | ct = (2*B/377)/((KV^2)/MVA);
      | ro = 2.5*R*(KV^2)/MVA;
      | lo = 2.5*(X/377)*(KV^2)/MVA;
      | co = (2*B/377)/((1.6*KV^2)/MVA);
      mask Display:
      | plot([0.2 0.8 0.8 0.2 0.2], [0.35 0.35 0.65 0.65 0.35]);
      | text(0.5, 0.5, 'π', 'horizontalAlignment', 'center');
  Line 19-20-2 : Subsystem  mask{R=0.017, X=0.034, B=2.5e-05, MVA=100, KV=33}
      mask prompts: R "Resistance (pu)"; X "Reactance(pu)"; B "Susceptance (pu)(B/2)"; MVA "MVA Base"; KV "KV Base"
      mask help: Transmission Line Pi model
      mask init:
      | rt = R*(KV^2)/MVA;
      | lt = (X/377)*(KV^2)/MVA;
      | ct = (2*B/377)/((KV^2)/MVA);
      | ro = 2.5*R*(KV^2)/MVA;
      | lo = 2.5*(X/377)*(KV^2)/MVA;
      | co = (2*B/377)/((1.6*KV^2)/MVA);
      mask Display:
      | plot([0.2 0.8 0.8 0.2 0.2], [0.35 0.35 0.65 0.65 0.35]);
      | text(0.5, 0.5, 'π', 'horizontalAlignment', 'center');
  Line 2-4-1 : Subsystem  mask{R=0.0285, X=0.087, B=0.0092, MVA=100, KV=132}
      mask prompts: R "Resistance (pu)"; X "Reactance(pu)"; B "Susceptance (pu)(B/2)"; MVA "MVA Base"; KV "KV Base"
      mask help: Transmission Line Pi model
      mask init:
      | rt = R*(KV^2)/MVA;
      | lt = (X/377)*(KV^2)/MVA;
      | ct = (2*B/377)/((KV^2)/MVA);
      | ro = 2.5*R*(KV^2)/MVA;
      | lo = 2.5*(X/377)*(KV^2)/MVA;
      | co = (2*B/377)/((1.6*KV^2)/MVA);
      mask Display:
      | plot([0.2 0.8 0.8 0.2 0.2], [0.35 0.35 0.65 0.65 0.35]);
      | text(0.5, 0.5, 'π', 'horizontalAlignment', 'center');
  Line 2-4-2 : Subsystem  mask{R=0.0285, X=0.087, B=0.0092, MVA=100, KV=132}
      mask prompts: R "Resistance (pu)"; X "Reactance(pu)"; B "Susceptance (pu)(B/2)"; MVA "MVA Base"; KV "KV Base"
      mask help: Transmission Line Pi model
      mask init:
      | rt = R*(KV^2)/MVA;
      | lt = (X/377)*(KV^2)/MVA;
      | ct = (2*B/377)/((KV^2)/MVA);
      | ro = 2.5*R*(KV^2)/MVA;
      | lo = 2.5*(X/377)*(KV^2)/MVA;
      | co = (2*B/377)/((1.6*KV^2)/MVA);
      mask Display:
      | plot([0.2 0.8 0.8 0.2 0.2], [0.35 0.35 0.65 0.65 0.35]);
      | text(0.5, 0.5, 'π', 'horizontalAlignment', 'center');
  Line 2-5-1 : Subsystem  mask{R=0.0236, X=0.099, B=0.0037, MVA=100, KV=132}
      mask prompts: R "Resistance (pu)"; X "Reactance(pu)"; B "Susceptance (pu)(B/2)"; MVA "MVA Base"; KV "KV Base"
      mask help: Transmission Line Pi model
      mask init:
      | rt = R*(KV^2)/MVA;
      | lt = (X/377)*(KV^2)/MVA;
      | ct = (2*B/377)/((KV^2)/MVA);
      | ro = 2.5*R*(KV^2)/MVA;
      | lo = 2.5*(X/377)*(KV^2)/MVA;
      | co = (2*B/377)/((1.6*KV^2)/MVA);
      mask Display:
      | plot([0.2 0.8 0.8 0.2 0.2], [0.35 0.35 0.65 0.65 0.35]);
      | text(0.5, 0.5, 'π', 'horizontalAlignment', 'center');
  Line 2-5-2 : Subsystem  mask{R=0.0236, X=0.099, B=0.0037, MVA=100, KV=132}
      mask prompts: R "Resistance (pu)"; X "Reactance(pu)"; B "Susceptance (pu)(B/2)"; MVA "MVA Base"; KV "KV Base"
      mask help: Transmission Line Pi model
      mask init:
      | rt = R*(KV^2)/MVA;
      | lt = (X/377)*(KV^2)/MVA;
      | ct = (2*B/377)/((KV^2)/MVA);
      | ro = 2.5*R*(KV^2)/MVA;
      | lo = 2.5*(X/377)*(KV^2)/MVA;
      | co = (2*B/377)/((1.6*KV^2)/MVA);
      mask Display:
      | plot([0.2 0.8 0.8 0.2 0.2], [0.35 0.35 0.65 0.65 0.35]);
      | text(0.5, 0.5, 'π', 'horizontalAlignment', 'center');
  Line 2-6-1 : Subsystem  mask{R=0.02905, X=0.088, B=0.00935, MVA=100, KV=132}
      mask prompts: R "Resistance (pu)"; X "Reactance(pu)"; B "Susceptance (pu)(B/2)"; MVA "MVA Base"; KV "KV Base"
      mask help: Transmission Line Pi model
      mask init:
      | rt = R*(KV^2)/MVA;
      | lt = (X/377)*(KV^2)/MVA;
      | ct = (2*B/377)/((KV^2)/MVA);
      | ro = 2.5*R*(KV^2)/MVA;
      | lo = 2.5*(X/377)*(KV^2)/MVA;
      | co = (2*B/377)/((1.6*KV^2)/MVA);
      mask Display:
      | plot([0.2 0.8 0.8 0.2 0.2], [0.35 0.35 0.65 0.65 0.35]);
      | text(0.5, 0.5, 'π', 'horizontalAlignment', 'center');
  Line 2-6-2 : Subsystem  mask{R=0.02905, X=0.088, B=0.00935, MVA=100, KV=132}
      mask prompts: R "Resistance (pu)"; X "Reactance(pu)"; B "Susceptance (pu)(B/2)"; MVA "MVA Base"; KV "KV Base"
      mask help: Transmission Line Pi model
      mask init:
      | rt = R*(KV^2)/MVA;
      | lt = (X/377)*(KV^2)/MVA;
      | ct = (2*B/377)/((KV^2)/MVA);
      | ro = 2.5*R*(KV^2)/MVA;
      | lo = 2.5*(X/377)*(KV^2)/MVA;
      | co = (2*B/377)/((1.6*KV^2)/MVA);
      mask Display:
      | plot([0.2 0.8 0.8 0.2 0.2], [0.35 0.35 0.65 0.65 0.35]);
      | text(0.5, 0.5, 'π', 'horizontalAlignment', 'center');
  Line 21-22-1 : Subsystem  mask{R=0.0058, X=0.118, B=2.5e-05, MVA=100, KV=33}
      mask prompts: R "Resistance (pu)"; X "Reactance(pu)"; B "Susceptance (pu)(B/2)"; MVA "MVA Base"; KV "KV Base"
      mask help: Transmission Line Pi model
      mask init:
      | rt = R*(KV^2)/MVA;
      | lt = (X/377)*(KV^2)/MVA;
      | ct = (2*B/377)/((KV^2)/MVA);
      | ro = 2.5*R*(KV^2)/MVA;
      | lo = 2.5*(X/377)*(KV^2)/MVA;
      | co = (2*B/377)/((1.6*KV^2)/MVA);
      mask Display:
      | plot([0.2 0.8 0.8 0.2 0.2], [0.35 0.35 0.65 0.65 0.35]);
      | text(0.5, 0.5, 'π', 'horizontalAlignment', 'center');
  Line 21-22-2 : Subsystem  mask{R=0.0058, X=0.118, B=2.5e-05, MVA=100, KV=33}
      mask prompts: R "Resistance (pu)"; X "Reactance(pu)"; B "Susceptance (pu)(B/2)"; MVA "MVA Base"; KV "KV Base"
      mask help: Transmission Line Pi model
      mask init:
      | rt = R*(KV^2)/MVA;
      | lt = (X/377)*(KV^2)/MVA;
      | ct = (2*B/377)/((KV^2)/MVA);
      | ro = 2.5*R*(KV^2)/MVA;
      | lo = 2.5*(X/377)*(KV^2)/MVA;
      | co = (2*B/377)/((1.6*KV^2)/MVA);
      mask Display:
      | plot([0.2 0.8 0.8 0.2 0.2], [0.35 0.35 0.65 0.65 0.35]);
      | text(0.5, 0.5, 'π', 'horizontalAlignment', 'center');
  Line 22-24-1 : Subsystem  mask{R=0.0575, X=0.0895, B=2.5e-05, MVA=100, KV=33}
      mask prompts: R "Resistance (pu)"; X "Reactance(pu)"; B "Susceptance (pu)(B/2)"; MVA "MVA Base"; KV "KV Base"
      mask help: Transmission Line Pi model
      mask init:
      | rt = R*(KV^2)/MVA;
      | lt = (X/377)*(KV^2)/MVA;
      | ct = (2*B/377)/((KV^2)/MVA);
      | ro = 2.5*R*(KV^2)/MVA;
      | lo = 2.5*(X/377)*(KV^2)/MVA;
      | co = (2*B/377)/((1.6*KV^2)/MVA);
      mask Display:
      | plot([0.2 0.8 0.8 0.2 0.2], [0.35 0.35 0.65 0.65 0.35]);
      | text(0.5, 0.5, 'π', 'horizontalAlignment', 'center');
  Line 22-24-2 : Subsystem  mask{R=0.0575, X=0.0895, B=2.5e-05, MVA=100, KV=33}
      mask prompts: R "Resistance (pu)"; X "Reactance(pu)"; B "Susceptance (pu)(B/2)"; MVA "MVA Base"; KV "KV Base"
      mask help: Transmission Line Pi model
      mask init:
      | rt = R*(KV^2)/MVA;
      | lt = (X/377)*(KV^2)/MVA;
      | ct = (2*B/377)/((KV^2)/MVA);
      | ro = 2.5*R*(KV^2)/MVA;
      | lo = 2.5*(X/377)*(KV^2)/MVA;
      | co = (2*B/377)/((1.6*KV^2)/MVA);
      mask Display:
      | plot([0.2 0.8 0.8 0.2 0.2], [0.35 0.35 0.65 0.65 0.35]);
      | text(0.5, 0.5, 'π', 'horizontalAlignment', 'center');
  Line 23-24-1 : Subsystem  mask{R=0.066, X=0.135, B=2.5e-05, MVA=100, KV=33}
      mask prompts: R "Resistance (pu)"; X "Reactance(pu)"; B "Susceptance (pu)(B/2)"; MVA "MVA Base"; KV "KV Base"
      mask help: Transmission Line Pi model
      mask init:
      | rt = R*(KV^2)/MVA;
      | lt = (X/377)*(KV^2)/MVA;
      | ct = (2*B/377)/((KV^2)/MVA);
      | ro = 2.5*R*(KV^2)/MVA;
      | lo = 2.5*(X/377)*(KV^2)/MVA;
      | co = (2*B/377)/((1.6*KV^2)/MVA);
      mask Display:
      | plot([0.2 0.8 0.8 0.2 0.2], [0.35 0.35 0.65 0.65 0.35]);
      | text(0.5, 0.5, 'π', 'horizontalAlignment', 'center');
  Line 23-24-2 : Subsystem  mask{R=0.066, X=0.135, B=2.5e-05, MVA=100, KV=33}
      mask prompts: R "Resistance (pu)"; X "Reactance(pu)"; B "Susceptance (pu)(B/2)"; MVA "MVA Base"; KV "KV Base"
      mask help: Transmission Line Pi model
      mask init:
      | rt = R*(KV^2)/MVA;
      | lt = (X/377)*(KV^2)/MVA;
      | ct = (2*B/377)/((KV^2)/MVA);
      | ro = 2.5*R*(KV^2)/MVA;
      | lo = 2.5*(X/377)*(KV^2)/MVA;
      | co = (2*B/377)/((1.6*KV^2)/MVA);
      mask Display:
      | plot([0.2 0.8 0.8 0.2 0.2], [0.35 0.35 0.65 0.65 0.35]);
      | text(0.5, 0.5, 'π', 'horizontalAlignment', 'center');
  Line 24-25-1 : Subsystem  mask{R=0.0945, X=0.1645, B=2.5e-05, MVA=100, KV=33}
      mask prompts: R "Resistance (pu)"; X "Reactance(pu)"; B "Susceptance (pu)(B/2)"; MVA "MVA Base"; KV "KV Base"
      mask help: Transmission Line Pi model
      mask init:
      | rt = R*(KV^2)/MVA;
      | lt = (X/377)*(KV^2)/MVA;
      | ct = (2*B/377)/((KV^2)/MVA);
      | ro = 2.5*R*(KV^2)/MVA;
      | lo = 2.5*(X/377)*(KV^2)/MVA;
      | co = (2*B/377)/((1.6*KV^2)/MVA);
      mask Display:
      | plot([0.2 0.8 0.8 0.2 0.2], [0.35 0.35 0.65 0.65 0.35]);
      | text(0.5, 0.5, 'π', 'horizontalAlignment', 'center');
  Line 24-25-2 : Subsystem  mask{R=0.0945, X=0.1645, B=2.5e-05, MVA=100, KV=33}
      mask prompts: R "Resistance (pu)"; X "Reactance(pu)"; B "Susceptance (pu)(B/2)"; MVA "MVA Base"; KV "KV Base"
      mask help: Transmission Line Pi model
      mask init:
      | rt = R*(KV^2)/MVA;
      | lt = (X/377)*(KV^2)/MVA;
      | ct = (2*B/377)/((KV^2)/MVA);
      | ro = 2.5*R*(KV^2)/MVA;
      | lo = 2.5*(X/377)*(KV^2)/MVA;
      | co = (2*B/377)/((1.6*KV^2)/MVA);
      mask Display:
      | plot([0.2 0.8 0.8 0.2 0.2], [0.35 0.35 0.65 0.65 0.35]);
      | text(0.5, 0.5, 'π', 'horizontalAlignment', 'center');
  Line 25-26-1 : Subsystem  mask{R=0.127, X=0.19, B=2.5e-05, MVA=100, KV=33}
      mask prompts: R "Resistance (pu)"; X "Reactance(pu)"; B "Susceptance (pu)(B/2)"; MVA "MVA Base"; KV "KV Base"
      mask help: Transmission Line Pi model
      mask init:
      | rt = R*(KV^2)/MVA;
      | lt = (X/377)*(KV^2)/MVA;
      | ct = (2*B/377)/((KV^2)/MVA);
      | ro = 2.5*R*(KV^2)/MVA;
      | lo = 2.5*(X/377)*(KV^2)/MVA;
      | co = (2*B/377)/((1.6*KV^2)/MVA);
      mask Display:
      | plot([0.2 0.8 0.8 0.2 0.2], [0.35 0.35 0.65 0.65 0.35]);
      | text(0.5, 0.5, 'π', 'horizontalAlignment', 'center');
  Line 25-26-2 : Subsystem  mask{R=0.127, X=0.19, B=2.5e-05, MVA=100, KV=33}
      mask prompts: R "Resistance (pu)"; X "Reactance(pu)"; B "Susceptance (pu)(B/2)"; MVA "MVA Base"; KV "KV Base"
      mask help: Transmission Line Pi model
      mask init:
      | rt = R*(KV^2)/MVA;
      | lt = (X/377)*(KV^2)/MVA;
      | ct = (2*B/377)/((KV^2)/MVA);
      | ro = 2.5*R*(KV^2)/MVA;
      | lo = 2.5*(X/377)*(KV^2)/MVA;
      | co = (2*B/377)/((1.6*KV^2)/MVA);
      mask Display:
      | plot([0.2 0.8 0.8 0.2 0.2], [0.35 0.35 0.65 0.65 0.35]);
      | text(0.5, 0.5, 'π', 'horizontalAlignment', 'center');
  Line 25-27-1 : Subsystem  mask{R=0.0545, X=0.1045, B=2.5e-05, MVA=100, KV=33}
      mask prompts: R "Resistance (pu)"; X "Reactance(pu)"; B "Susceptance (pu)(B/2)"; MVA "MVA Base"; KV "KV Base"
      mask help: Transmission Line Pi model
      mask init:
      | rt = R*(KV^2)/MVA;
      | lt = (X/377)*(KV^2)/MVA;
      | ct = (2*B/377)/((KV^2)/MVA);
      | ro = 2.5*R*(KV^2)/MVA;
      | lo = 2.5*(X/377)*(KV^2)/MVA;
      | co = (2*B/377)/((1.6*KV^2)/MVA);
      mask Display:
      | plot([0.2 0.8 0.8 0.2 0.2], [0.35 0.35 0.65 0.65 0.35]);
      | text(0.5, 0.5, 'π', 'horizontalAlignment', 'center');
  Line 25-27-2 : Subsystem  mask{R=0.0545, X=0.1045, B=2.5e-05, MVA=100, KV=33}
      mask prompts: R "Resistance (pu)"; X "Reactance(pu)"; B "Susceptance (pu)(B/2)"; MVA "MVA Base"; KV "KV Base"
      mask help: Transmission Line Pi model
      mask init:
      | rt = R*(KV^2)/MVA;
      | lt = (X/377)*(KV^2)/MVA;
      | ct = (2*B/377)/((KV^2)/MVA);
      | ro = 2.5*R*(KV^2)/MVA;
      | lo = 2.5*(X/377)*(KV^2)/MVA;
      | co = (2*B/377)/((1.6*KV^2)/MVA);
      mask Display:
      | plot([0.2 0.8 0.8 0.2 0.2], [0.35 0.35 0.65 0.65 0.35]);
      | text(0.5, 0.5, 'π', 'horizontalAlignment', 'center');
  Line 27-29-1 : Subsystem  mask{R=0.11, X=0.2075, B=2.5e-05, MVA=100, KV=33}
      mask prompts: R "Resistance (pu)"; X "Reactance(pu)"; B "Susceptance (pu)(B/2)"; MVA "MVA Base"; KV "KV Base"
      mask help: Transmission Line Pi model
      mask init:
      | rt = R*(KV^2)/MVA;
      | lt = (X/377)*(KV^2)/MVA;
      | ct = (2*B/377)/((KV^2)/MVA);
      | ro = 2.5*R*(KV^2)/MVA;
      | lo = 2.5*(X/377)*(KV^2)/MVA;
      | co = (2*B/377)/((1.6*KV^2)/MVA);
      mask Display:
      | plot([0.2 0.8 0.8 0.2 0.2], [0.35 0.35 0.65 0.65 0.35]);
      | text(0.5, 0.5, 'π', 'horizontalAlignment', 'center');
  Line 27-29-2 : Subsystem  mask{R=0.11, X=0.2075, B=2.5e-05, MVA=100, KV=33}
      mask prompts: R "Resistance (pu)"; X "Reactance(pu)"; B "Susceptance (pu)(B/2)"; MVA "MVA Base"; KV "KV Base"
      mask help: Transmission Line Pi model
      mask init:
      | rt = R*(KV^2)/MVA;
      | lt = (X/377)*(KV^2)/MVA;
      | ct = (2*B/377)/((KV^2)/MVA);
      | ro = 2.5*R*(KV^2)/MVA;
      | lo = 2.5*(X/377)*(KV^2)/MVA;
      | co = (2*B/377)/((1.6*KV^2)/MVA);
      mask Display:
      | plot([0.2 0.8 0.8 0.2 0.2], [0.35 0.35 0.65 0.65 0.35]);
      | text(0.5, 0.5, 'π', 'horizontalAlignment', 'center');
  Line 27-30-1 : Subsystem  mask{R=0.16, X=0.3015, B=2.5e-05, MVA=100, KV=33}
      mask prompts: R "Resistance (pu)"; X "Reactance(pu)"; B "Susceptance (pu)(B/2)"; MVA "MVA Base"; KV "KV Base"
      mask help: Transmission Line Pi model
      mask init:
      | rt = R*(KV^2)/MVA;
      | lt = (X/377)*(KV^2)/MVA;
      | ct = (2*B/377)/((KV^2)/MVA);
      | ro = 2.5*R*(KV^2)/MVA;
      | lo = 2.5*(X/377)*(KV^2)/MVA;
      | co = (2*B/377)/((1.6*KV^2)/MVA);
      mask Display:
      | plot([0.2 0.8 0.8 0.2 0.2], [0.35 0.35 0.65 0.65 0.35]);
      | text(0.5, 0.5, 'π', 'horizontalAlignment', 'center');
  Line 27-30-2 : Subsystem  mask{R=0.16, X=0.3015, B=2.5e-05, MVA=100, KV=33}
      mask prompts: R "Resistance (pu)"; X "Reactance(pu)"; B "Susceptance (pu)(B/2)"; MVA "MVA Base"; KV "KV Base"
      mask help: Transmission Line Pi model
      mask init:
      | rt = R*(KV^2)/MVA;
      | lt = (X/377)*(KV^2)/MVA;
      | ct = (2*B/377)/((KV^2)/MVA);
      | ro = 2.5*R*(KV^2)/MVA;
      | lo = 2.5*(X/377)*(KV^2)/MVA;
      | co = (2*B/377)/((1.6*KV^2)/MVA);
      mask Display:
      | plot([0.2 0.8 0.8 0.2 0.2], [0.35 0.35 0.65 0.65 0.35]);
      | text(0.5, 0.5, 'π', 'horizontalAlignment', 'center');
  Line 29-30-1 : Subsystem  mask{R=0.12, X=0.2265, B=2.5e-05, MVA=100, KV=33}
      mask prompts: R "Resistance (pu)"; X "Reactance(pu)"; B "Susceptance (pu)(B/2)"; MVA "MVA Base"; KV "KV Base"
      mask help: Transmission Line Pi model
      mask init:
      | rt = R*(KV^2)/MVA;
      | lt = (X/377)*(KV^2)/MVA;
      | ct = (2*B/377)/((KV^2)/MVA);
      | ro = 2.5*R*(KV^2)/MVA;
      | lo = 2.5*(X/377)*(KV^2)/MVA;
      | co = (2*B/377)/((1.6*KV^2)/MVA);
      mask Display:
      | plot([0.2 0.8 0.8 0.2 0.2], [0.35 0.35 0.65 0.65 0.35]);
      | text(0.5, 0.5, 'π', 'horizontalAlignment', 'center');
  Line 29-30-2 : Subsystem  mask{R=0.12, X=0.2265, B=2.5e-05, MVA=100, KV=33}
      mask prompts: R "Resistance (pu)"; X "Reactance(pu)"; B "Susceptance (pu)(B/2)"; MVA "MVA Base"; KV "KV Base"
      mask help: Transmission Line Pi model
      mask init:
      | rt = R*(KV^2)/MVA;
      | lt = (X/377)*(KV^2)/MVA;
      | ct = (2*B/377)/((KV^2)/MVA);
      | ro = 2.5*R*(KV^2)/MVA;
      | lo = 2.5*(X/377)*(KV^2)/MVA;
      | co = (2*B/377)/((1.6*KV^2)/MVA);
      mask Display:
      | plot([0.2 0.8 0.8 0.2 0.2], [0.35 0.35 0.65 0.65 0.35]);
      | text(0.5, 0.5, 'π', 'horizontalAlignment', 'center');
  Line 3-4-1 : Subsystem  mask{R=0.0066, X=0.01895, B=0.0021, MVA=100, KV=132}
      mask prompts: R "Resistance (pu)"; X "Reactance(pu)"; B "Susceptance (pu)(B/2)"; MVA "MVA Base"; KV "KV Base"
      mask help: Transmission Line Pi model
      mask init:
      | rt = R*(KV^2)/MVA;
      | lt = (X/377)*(KV^2)/MVA;
      | ct = (2*B/377)/((KV^2)/MVA);
      | ro = 2.5*R*(KV^2)/MVA;
      | lo = 2.5*(X/377)*(KV^2)/MVA;
      | co = (2*B/377)/((1.6*KV^2)/MVA);
      mask Display:
      | plot([0.2 0.8 0.8 0.2 0.2], [0.35 0.35 0.65 0.65 0.35]);
      | text(0.5, 0.5, 'π', 'horizontalAlignment', 'center');
  Line 3-4-2 : Subsystem  mask{R=0.0066, X=0.01895, B=0.0021, MVA=100, KV=132}
      mask prompts: R "Resistance (pu)"; X "Reactance(pu)"; B "Susceptance (pu)(B/2)"; MVA "MVA Base"; KV "KV Base"
      mask help: Transmission Line Pi model
      mask init:
      | rt = R*(KV^2)/MVA;
      | lt = (X/377)*(KV^2)/MVA;
      | ct = (2*B/377)/((KV^2)/MVA);
      | ro = 2.5*R*(KV^2)/MVA;
      | lo = 2.5*(X/377)*(KV^2)/MVA;
      | co = (2*B/377)/((1.6*KV^2)/MVA);
      mask Display:
      | plot([0.2 0.8 0.8 0.2 0.2], [0.35 0.35 0.65 0.65 0.35]);
      | text(0.5, 0.5, 'π', 'horizontalAlignment', 'center');
  Line 4-6-1 : Subsystem  mask{R=0.00595, X=0.0207, B=0.00225, MVA=100, KV=132}
      mask prompts: R "Resistance (pu)"; X "Reactance(pu)"; B "Susceptance (pu)(B/2)"; MVA "MVA Base"; KV "KV Base"
      mask help: Transmission Line Pi model
      mask init:
      | rt = R*(KV^2)/MVA;
      | lt = (X/377)*(KV^2)/MVA;
      | ct = (2*B/377)/((KV^2)/MVA);
      | ro = 2.5*R*(KV^2)/MVA;
      | lo = 2.5*(X/377)*(KV^2)/MVA;
      | co = (2*B/377)/((1.6*KV^2)/MVA);
      mask Display:
      | plot([0.2 0.8 0.8 0.2 0.2], [0.35 0.35 0.65 0.65 0.35]);
      | text(0.5, 0.5, 'π', 'horizontalAlignment', 'center');
  Line 4-6-2 : Subsystem  mask{R=0.00595, X=0.0207, B=0.00225, MVA=100, KV=132}
      mask prompts: R "Resistance (pu)"; X "Reactance(pu)"; B "Susceptance (pu)(B/2)"; MVA "MVA Base"; KV "KV Base"
      mask help: Transmission Line Pi model
      mask init:
      | rt = R*(KV^2)/MVA;
      | lt = (X/377)*(KV^2)/MVA;
      | ct = (2*B/377)/((KV^2)/MVA);
      | ro = 2.5*R*(KV^2)/MVA;
      | lo = 2.5*(X/377)*(KV^2)/MVA;
      | co = (2*B/377)/((1.6*KV^2)/MVA);
      mask Display:
      | plot([0.2 0.8 0.8 0.2 0.2], [0.35 0.35 0.65 0.65 0.35]);
      | text(0.5, 0.5, 'π', 'horizontalAlignment', 'center');
  Line 5-7-1 : Subsystem  mask{R=0.023, X=0.058, B=0.0051, MVA=100, KV=132}
      mask prompts: R "Resistance (pu)"; X "Reactance(pu)"; B "Susceptance (pu)(B/2)"; MVA "MVA Base"; KV "KV Base"
      mask help: Transmission Line Pi model
      mask init:
      | rt = R*(KV^2)/MVA;
      | lt = (X/377)*(KV^2)/MVA;
      | ct = (2*B/377)/((KV^2)/MVA);
      | ro = 2.5*R*(KV^2)/MVA;
      | lo = 2.5*(X/377)*(KV^2)/MVA;
      | co = (2*B/377)/((1.6*KV^2)/MVA);
      mask Display:
      | plot([0.2 0.8 0.8 0.2 0.2], [0.35 0.35 0.65 0.65 0.35]);
      | text(0.5, 0.5, 'π', 'horizontalAlignment', 'center');
  Line 5-7-2 : Subsystem  mask{R=0.023, X=0.058, B=0.0051, MVA=100, KV=132}
      mask prompts: R "Resistance (pu)"; X "Reactance(pu)"; B "Susceptance (pu)(B/2)"; MVA "MVA Base"; KV "KV Base"
      mask help: Transmission Line Pi model
      mask init:
      | rt = R*(KV^2)/MVA;
      | lt = (X/377)*(KV^2)/MVA;
      | ct = (2*B/377)/((KV^2)/MVA);
      | ro = 2.5*R*(KV^2)/MVA;
      | lo = 2.5*(X/377)*(KV^2)/MVA;
      | co = (2*B/377)/((1.6*KV^2)/MVA);
      mask Display:
      | plot([0.2 0.8 0.8 0.2 0.2], [0.35 0.35 0.65 0.65 0.35]);
      | text(0.5, 0.5, 'π', 'horizontalAlignment', 'center');
  Line 6-28-1 : Subsystem  mask{R=0.00845, X=0.02995, B=0.00325, MVA=100, KV=132}
      mask prompts: R "Resistance (pu)"; X "Reactance(pu)"; B "Susceptance (pu)(B/2)"; MVA "MVA Base"; KV "KV Base"
      mask help: Transmission Line Pi model
      mask init:
      | rt = R*(KV^2)/MVA;
      | lt = (X/377)*(KV^2)/MVA;
      | ct = (2*B/377)/((KV^2)/MVA);
      | ro = 2.5*R*(KV^2)/MVA;
      | lo = 2.5*(X/377)*(KV^2)/MVA;
      | co = (2*B/377)/((1.6*KV^2)/MVA);
      mask Display:
      | plot([0.2 0.8 0.8 0.2 0.2], [0.35 0.35 0.65 0.65 0.35]);
      | text(0.5, 0.5, 'π', 'horizontalAlignment', 'center');
  Line 6-28-2 : Subsystem  mask{R=0.00845, X=0.02995, B=0.00325, MVA=100, KV=132}
      mask prompts: R "Resistance (pu)"; X "Reactance(pu)"; B "Susceptance (pu)(B/2)"; MVA "MVA Base"; KV "KV Base"
      mask help: Transmission Line Pi model
      mask init:
      | rt = R*(KV^2)/MVA;
      | lt = (X/377)*(KV^2)/MVA;
      | ct = (2*B/377)/((KV^2)/MVA);
      | ro = 2.5*R*(KV^2)/MVA;
      | lo = 2.5*(X/377)*(KV^2)/MVA;
      | co = (2*B/377)/((1.6*KV^2)/MVA);
      mask Display:
      | plot([0.2 0.8 0.8 0.2 0.2], [0.35 0.35 0.65 0.65 0.35]);
      | text(0.5, 0.5, 'π', 'horizontalAlignment', 'center');
  Line 6-7-1 : Subsystem  mask{R=0.01335, X=0.041, B=0.00425, MVA=100, KV=132}
      mask prompts: R "Resistance (pu)"; X "Reactance(pu)"; B "Susceptance (pu)(B/2)"; MVA "MVA Base"; KV "KV Base"
      mask help: Transmission Line Pi model
      mask init:
      | rt = R*(KV^2)/MVA;
      | lt = (X/377)*(KV^2)/MVA;
      | ct = (2*B/377)/((KV^2)/MVA);
      | ro = 2.5*R*(KV^2)/MVA;
      | lo = 2.5*(X/377)*(KV^2)/MVA;
      | co = (2*B/377)/((1.6*KV^2)/MVA);
      mask Display:
      | plot([0.2 0.8 0.8 0.2 0.2], [0.35 0.35 0.65 0.65 0.35]);
      | text(0.5, 0.5, 'π', 'horizontalAlignment', 'center');
  Line 6-7-2 : Subsystem  mask{R=0.01335, X=0.041, B=0.00425, MVA=100, KV=132}
      mask prompts: R "Resistance (pu)"; X "Reactance(pu)"; B "Susceptance (pu)(B/2)"; MVA "MVA Base"; KV "KV Base"
      mask help: Transmission Line Pi model
      mask init:
      | rt = R*(KV^2)/MVA;
      | lt = (X/377)*(KV^2)/MVA;
      | ct = (2*B/377)/((KV^2)/MVA);
      | ro = 2.5*R*(KV^2)/MVA;
      | lo = 2.5*(X/377)*(KV^2)/MVA;
      | co = (2*B/377)/((1.6*KV^2)/MVA);
      mask Display:
      | plot([0.2 0.8 0.8 0.2 0.2], [0.35 0.35 0.65 0.65 0.35]);
      | text(0.5, 0.5, 'π', 'horizontalAlignment', 'center');
  Line 6-8-1 : Subsystem  mask{R=0.006, X=0.021, B=0.00225, MVA=100, KV=132}
      mask prompts: R "Resistance (pu)"; X "Reactance(pu)"; B "Susceptance (pu)(B/2)"; MVA "MVA Base"; KV "KV Base"
      mask help: Transmission Line Pi model
      mask init:
      | rt = R*(KV^2)/MVA;
      | lt = (X/377)*(KV^2)/MVA;
      | ct = (2*B/377)/((KV^2)/MVA);
      | ro = 2.5*R*(KV^2)/MVA;
      | lo = 2.5*(X/377)*(KV^2)/MVA;
      | co = (2*B/377)/((1.6*KV^2)/MVA);
      mask Display:
      | plot([0.2 0.8 0.8 0.2 0.2], [0.35 0.35 0.65 0.65 0.35]);
      | text(0.5, 0.5, 'π', 'horizontalAlignment', 'center');
  Line 6-8-2 : Subsystem  mask{R=0.006, X=0.021, B=0.00225, MVA=100, KV=132}
      mask prompts: R "Resistance (pu)"; X "Reactance(pu)"; B "Susceptance (pu)(B/2)"; MVA "MVA Base"; KV "KV Base"
      mask help: Transmission Line Pi model
      mask init:
      | rt = R*(KV^2)/MVA;
      | lt = (X/377)*(KV^2)/MVA;
      | ct = (2*B/377)/((KV^2)/MVA);
      | ro = 2.5*R*(KV^2)/MVA;
      | lo = 2.5*(X/377)*(KV^2)/MVA;
      | co = (2*B/377)/((1.6*KV^2)/MVA);
      mask Display:
      | plot([0.2 0.8 0.8 0.2 0.2], [0.35 0.35 0.65 0.65 0.35]);
      | text(0.5, 0.5, 'π', 'horizontalAlignment', 'center');
  Line 8-28-1 : Subsystem  mask{R=0.0318, X=0.1, B=0.0107, MVA=100, KV=132}
      mask prompts: R "Resistance (pu)"; X "Reactance(pu)"; B "Susceptance (pu)(B/2)"; MVA "MVA Base"; KV "KV Base"
      mask help: Transmission Line Pi model
      mask init:
      | rt = R*(KV^2)/MVA;
      | lt = (X/377)*(KV^2)/MVA;
      | ct = (2*B/377)/((KV^2)/MVA);
      | ro = 2.5*R*(KV^2)/MVA;
      | lo = 2.5*(X/377)*(KV^2)/MVA;
      | co = (2*B/377)/((1.6*KV^2)/MVA);
      mask Display:
      | plot([0.2 0.8 0.8 0.2 0.2], [0.35 0.35 0.65 0.65 0.35]);
      | text(0.5, 0.5, 'π', 'horizontalAlignment', 'center');
  Line 8-28-2 : Subsystem  mask{R=0.0318, X=0.1, B=0.0107, MVA=100, KV=132}
      mask prompts: R "Resistance (pu)"; X "Reactance(pu)"; B "Susceptance (pu)(B/2)"; MVA "MVA Base"; KV "KV Base"
      mask help: Transmission Line Pi model
      mask init:
      | rt = R*(KV^2)/MVA;
      | lt = (X/377)*(KV^2)/MVA;
      | ct = (2*B/377)/((KV^2)/MVA);
      | ro = 2.5*R*(KV^2)/MVA;
      | lo = 2.5*(X/377)*(KV^2)/MVA;
      | co = (2*B/377)/((1.6*KV^2)/MVA);
      mask Display:
      | plot([0.2 0.8 0.8 0.2 0.2], [0.35 0.35 0.65 0.65 0.35]);
      | text(0.5, 0.5, 'π', 'horizontalAlignment', 'center');
  Load Flow Bus1 : powerlib/Measurements/Load Flow Bus  LConnTagsString=a  Phases=single  Connectors=on one side  ID=BUS_2  Vbase=132e3  Vref=1.043  Vangle=0  VLF=1.019  VLFb=1  VLFc=1  angleLF=-5.131  angleLFb=0  angleLFc=0
      settings: AttributesFormatString=%<ID>\n%<Vbase>V\n%<VLF>pu\n%<angleLF>deg.  SourceProductName=Simscape Power Systems
  Load Flow Bus10 : powerlib/Measurements/Load Flow Bus  LConnTagsString=a  Phases=single  Connectors=on one side  ID=BUS_10  Vbase=33e3  Vref=1.045  Vangle=0  VLF=0.8361  VLFb=1  VLFc=1  angleLF=-20.87  angleLFb=0  angleLFc=0
      settings: AttributesFormatString=%<ID>\n%<Vbase>V\n%<VLF>pu\n%<angleLF>deg.  SourceProductName=Simscape Power Systems
  Load Flow Bus11 : powerlib/Measurements/Load Flow Bus  LConnTagsString=a  Phases=single  Connectors=on one side  ID=BUS_11  Vbase=33e3  Vref=1.082  Vangle=0  VLF=1.082  VLFb=1  VLFc=1  angleLF=-11.17  angleLFb=0  angleLFc=0
      settings: AttributesFormatString=%<ID>\n%<Vbase>V\n%<VLF>pu\n%<angleLF>deg.  SourceProductName=Simscape Power Systems
  Load Flow Bus12 : powerlib/Measurements/Load Flow Bus  LConnTagsString=a  Phases=single  Connectors=on one side  ID=BUS_12  Vbase=33e3  Vref=1.057  Vangle=0  VLF=0.8804  VLFb=1  VLFc=1  angleLF=-18.34  angleLFb=0  angleLFc=0
      settings: AttributesFormatString=%<ID>\n%<Vbase>V\n%<VLF>pu\n%<angleLF>deg.  SourceProductName=Simscape Power Systems
  Load Flow Bus13 : powerlib/Measurements/Load Flow Bus  LConnTagsString=a  Phases=single  Connectors=on one side  ID=BUS_13  Vbase=33e3  Vref=1.071  Vangle=0  VLF=1.071  VLFb=1  VLFc=1  angleLF=-18.34  angleLFb=0  angleLFc=0
      settings: AttributesFormatString=%<ID>\n%<Vbase>V\n%<VLF>pu\n%<angleLF>deg.  SourceProductName=Simscape Power Systems
  Load Flow Bus14 : powerlib/Measurements/Load Flow Bus  LConnTagsString=a  Phases=single  Connectors=on one side  ID=BUS_14  Vbase=33e3  Vref=1.042  Vangle=0  VLF=0.8599  VLFb=1  VLFc=1  angleLF=-19.76  angleLFb=0  angleLFc=0
      settings: AttributesFormatString=%<ID>\n%<Vbase>V\n%<VLF>pu\n%<angleLF>deg.  SourceProductName=Simscape Power Systems
  Load Flow Bus15 : powerlib/Measurements/Load Flow Bus  LConnTagsString=a  Phases=single  Connectors=on one side  ID=BUS_15  Vbase=33e3  Vref=1.038  Vangle=0  VLF=0.8512  VLFb=1  VLFc=1  angleLF=-19.95  angleLFb=0  angleLFc=0
      settings: AttributesFormatString=%<ID>\n%<Vbase>V\n%<VLF>pu\n%<angleLF>deg.  SourceProductName=Simscape Power Systems
  Load Flow Bus16 : powerlib/Measurements/Load Flow Bus  LConnTagsString=a  Phases=single  Connectors=on one side  ID=BUS_16  Vbase=33e3  Vref=1.045  Vangle=0  VLF=0.851  VLFb=1  VLFc=1  angleLF=-19.72  angleLFb=0  angleLFc=0
      settings: AttributesFormatString=%<ID>\n%<Vbase>V\n%<VLF>pu\n%<angleLF>deg.  SourceProductName=Simscape Power Systems
  Load Flow Bus17 : powerlib/Measurements/Load Flow Bus  LConnTagsString=a  Phases=single  Connectors=on one side  ID=BUS_17  Vbase=33e3  Vref=1.04  Vangle=0  VLF=0.8348  VLFb=1  VLFc=1  angleLF=-20.87  angleLFb=0  angleLFc=0
      settings: AttributesFormatString=%<ID>\n%<Vbase>V\n%<VLF>pu\n%<angleLF>deg.  SourceProductName=Simscape Power Systems
  Load Flow Bus18 : powerlib/Measurements/Load Flow Bus  LConnTagsString=a  Phases=single  Connectors=on one side  ID=BUS_18  Vbase=33e3  Vref=1.028  Vangle=0  VLF=0.8306  VLFb=1  VLFc=1  angleLF=-21.33  angleLFb=0  angleLFc=0
      settings: AttributesFormatString=%<ID>\n%<Vbase>V\n%<VLF>pu\n%<angleLF>deg.  SourceProductName=Simscape Power Systems
  Load Flow Bus19 : powerlib/Measurements/Load Flow Bus  LConnTagsString=a  Phases=single  Connectors=on one side  ID=BUS_19  Vbase=33e3  Vref=1.026  Vangle=0  VLF=0.8224  VLFb=1  VLFc=1  angleLF=-21.87  angleLFb=0  angleLFc=0
      settings: AttributesFormatString=%<ID>\n%<Vbase>V\n%<VLF>pu\n%<angleLF>deg.  SourceProductName=Simscape Power Systems
  Load Flow Bus2 : powerlib/Measurements/Load Flow Bus  LConnTagsString=a  Phases=single  Connectors=on one side  ID=BUS_3  Vbase=132e3  Vref=1.021  Vangle=0  VLF=0.98  VLFb=1  VLFc=1  angleLF=-7.295  angleLFb=0  angleLFc=0
      settings: AttributesFormatString=%<ID>\n%<Vbase>V\n%<VLF>pu\n%<angleLF>deg.  SourceProductName=Simscape Power Systems
  Load Flow Bus20 : powerlib/Measurements/Load Flow Bus  LConnTagsString=a  Phases=single  Connectors=on one side  ID=BUS_20  Vbase=33e3  Vref=1.03  Vangle=0  VLF=0.8248  VLFb=1  VLFc=1  angleLF=-21.71  angleLFb=0  angleLFc=0
      settings: AttributesFormatString=%<ID>\n%<Vbase>V\n%<VLF>pu\n%<angleLF>deg.  SourceProductName=Simscape Power Systems
  Load Flow Bus21 : powerlib/Measurements/Load Flow Bus  LConnTagsString=a  Phases=single  Connectors=on one side  ID=BUS_21  Vbase=33e3  Vref=1.033  Vangle=0  VLF=0.8217  VLFb=1  VLFc=1  angleLF=-21.52  angleLFb=0  angleLFc=0
      settings: AttributesFormatString=%<ID>\n%<Vbase>V\n%<VLF>pu\n%<angleLF>deg.  SourceProductName=Simscape Power Systems
  Load Flow Bus22 : powerlib/Measurements/Load Flow Bus  LConnTagsString=a  Phases=single  Connectors=on one side  ID=BUS_22  Vbase=33e3  Vref=1.033  Vangle=0  VLF=0.8285  VLFb=1  VLFc=1  angleLF=-20.96  angleLFb=0  angleLFc=0
      settings: AttributesFormatString=%<ID>\n%<Vbase>V\n%<VLF>pu\n%<angleLF>deg.  SourceProductName=Simscape Power Systems
  Load Flow Bus23 : powerlib/Measurements/Load Flow Bus  LConnTagsString=a  Phases=single  Connectors=on one side  ID=BUS_23  Vbase=33e3  Vref=1.027  Vangle=0  VLF=0.8366  VLFb=1  VLFc=1  angleLF=-20.53  angleLFb=0  angleLFc=0
      settings: AttributesFormatString=%<ID>\n%<Vbase>V\n%<VLF>pu\n%<angleLF>deg.  SourceProductName=Simscape Power Systems
  Load Flow Bus24 : powerlib/Measurements/Load Flow Bus  LConnTagsString=a  Phases=single  Connectors=on one side  ID=BUS_24  Vbase=33e3  Vref=1.021  Vangle=0  VLF=0.8274  VLFb=1  VLFc=1  angleLF=-20.78  angleLFb=0  angleLFc=0
      settings: AttributesFormatString=%<ID>\n%<Vbase>V\n%<VLF>pu\n%<angleLF>deg.  SourceProductName=Simscape Power Systems
  Load Flow Bus25 : powerlib/Measurements/Load Flow Bus  LConnTagsString=a  Phases=single  Connectors=on one side  ID=BUS_25  Vbase=33e3  Vref=1.017  Vangle=0  VLF=0.8603  VLFb=1  VLFc=1  angleLF=-19.43  angleLFb=0  angleLFc=0
      settings: AttributesFormatString=%<ID>\n%<Vbase>V\n%<VLF>pu\n%<angleLF>deg.  SourceProductName=Simscape Power Systems
  Load Flow Bus26 : powerlib/Measurements/Load Flow Bus  LConnTagsString=a  Phases=single  Connectors=on one side  ID=BUS_26  Vbase=33e3  Vref=1  Vangle=0  VLF=0.8392  VLFb=1  VLFc=1  angleLF=-20.02  angleLFb=0  angleLFc=0
      settings: AttributesFormatString=%<ID>\n%<Vbase>V\n%<VLF>pu\n%<angleLF>deg.  SourceProductName=Simscape Power Systems
  Load Flow Bus27 : powerlib/Measurements/Load Flow Bus  LConnTagsString=a  Phases=single  Connectors=on one side  ID=BUS_27  Vbase=33e3  Vref=1.023  Vangle=0  VLF=0.8908  VLFb=1  VLFc=1  angleLF=-18.23  angleLFb=0  angleLFc=0
      settings: AttributesFormatString=%<ID>\n%<Vbase>V\n%<VLF>pu\n%<angleLF>deg.  SourceProductName=Simscape Power Systems
  Load Flow Bus28 : powerlib/Measurements/Load Flow Bus  LConnTagsString=a  Phases=single  Connectors=on one side  ID=BUS_28  Vbase=132e3  Vref=1.007  Vangle=0  VLF=0.9445  VLFb=1  VLFc=1  angleLF=-11.54  angleLFb=0  angleLFc=0
      settings: AttributesFormatString=%<ID>\n%<Vbase>V\n%<VLF>pu\n%<angleLF>deg.  SourceProductName=Simscape Power Systems
  Load Flow Bus29 : powerlib/Measurements/Load Flow Bus  LConnTagsString=a  Phases=single  Connectors=on one side  ID=BUS_29  Vbase=33e3  Vref=1.003  Vangle=0  VLF=0.8676  VLFb=1  VLFc=1  angleLF=-19.87  angleLFb=0  angleLFc=0
      settings: AttributesFormatString=%<ID>\n%<Vbase>V\n%<VLF>pu\n%<angleLF>deg.  SourceProductName=Simscape Power Systems
  Load Flow Bus3 : powerlib/Measurements/Load Flow Bus  LConnTagsString=a  Phases=single  Connectors=on one side  ID=BUS_4  Vbase=132e3  Vref=1.012  Vangle=0  VLF=0.9614  VLFb=1  VLFc=1  angleLF=-9.041  angleLFb=0  angleLFc=0
      settings: AttributesFormatString=%<ID>\n%<Vbase>V\n%<VLF>pu\n%<angleLF>deg.  SourceProductName=Simscape Power Systems
  Load Flow Bus30 : powerlib/Measurements/Load Flow Bus  LConnTagsString=a  Phases=single  Connectors=on one side  ID=BUS_30  Vbase=33e3  Vref=0.992  Vangle=0  VLF=0.8542  VLFb=1  VLFc=1  angleLF=-21.05  angleLFb=0  angleLFc=0
      settings: AttributesFormatString=%<ID>\n%<Vbase>V\n%<VLF>pu\n%<angleLF>deg.  SourceProductName=Simscape Power Systems
  Load Flow Bus4 : powerlib/Measurements/Load Flow Bus  LConnTagsString=a  Phases=single  Connectors=on one side  ID=BUS_5  Vbase=132e3  Vref=1.01  Vangle=0  VLF=0.9703  VLFb=1  VLFc=1  angleLF=-14.42  angleLFb=0  angleLFc=0
      settings: AttributesFormatString=%<ID>\n%<Vbase>V\n%<VLF>pu\n%<angleLF>deg.  SourceProductName=Simscape Power Systems
  Load Flow Bus5 : powerlib/Measurements/Load Flow Bus  LConnTagsString=a  Phases=single  Connectors=on one side  ID=BUS_6  Vbase=132e3  Vref=1.01  Vangle=0  VLF=0.954  VLFb=1  VLFc=1  angleLF=-10.71  angleLFb=0  angleLFc=0
      settings: AttributesFormatString=%<ID>\n%<Vbase>V\n%<VLF>pu\n%<angleLF>deg.  SourceProductName=Simscape Power Systems
  Load Flow Bus6 : powerlib/Measurements/Load Flow Bus  LConnTagsString=a  Phases=single  Connectors=on one side  ID=BUS_7  Vbase=132e3  Vref=1.002  Vangle=0  VLF=0.9523  VLFb=1  VLFc=1  angleLF=-12.81  angleLFb=0  angleLFc=0
      settings: AttributesFormatString=%<ID>\n%<Vbase>V\n%<VLF>pu\n%<angleLF>deg.  SourceProductName=Simscape Power Systems
  Load Flow Bus7 : powerlib/Measurements/Load Flow Bus  LConnTagsString=a  Phases=single  Connectors=on one side  ID=BUS_1  Vbase=132e3  Vref=1.06  Vangle=0  VLF=1.06  VLFb=1  VLFc=1  angleLF=0  angleLFb=0  angleLFc=0
      settings: AttributesFormatString=%<ID>\n%<Vbase>V\n%<VLF>pu\n%<angleLF>deg.  SourceProductName=Simscape Power Systems
  Load Flow Bus8 : powerlib/Measurements/Load Flow Bus  LConnTagsString=a  Phases=single  Connectors=on one side  ID=BUS_8  Vbase=132e3  Vref=1.01  Vangle=0  VLF=0.9536  VLFb=1  VLFc=1  angleLF=-11.59  angleLFb=0  angleLFc=0
      settings: AttributesFormatString=%<ID>\n%<Vbase>V\n%<VLF>pu\n%<angleLF>deg.  SourceProductName=Simscape Power Systems
  Load Flow Bus9 : powerlib/Measurements/Load Flow Bus  LConnTagsString=a  Phases=single  Connectors=on one side  ID=BUS_9  Vbase=33e3  Vref=1.051  Vangle=0  VLF=0.9508  VLFb=1  VLFc=1  angleLF=-11.17  angleLFb=0  angleLFc=0
      settings: AttributesFormatString=%<ID>\n%<Vbase>V\n%<VLF>pu\n%<angleLF>deg.  SourceProductName=Simscape Power Systems
  Load10 : powerlib/Elements/Three-Phase Parallel RLC Load  LConnTagsString=A|B|C  Configuration=Y (grounded)  NominalVoltage=(33000)*0.836128  Vabc=[1e3 1e3 1e3]  Vabcp=[1e3 1e3 1e3]  NominalFrequency=60  UnbalancedPower=off  ActivePower=5.8e6  InductivePower=2e6  CapacitivePower=0  Pabc=[10e3 9e3 11e3]  QLabc=[100 90 110]  QCabc=[100 90 110]  Pabcp=[10e3 9e3 11e3]  QLabcp=[100 90 110]  QCabcp=[100 90 110]  Measurements=None  LoadType=constant PQ
  Load12 : powerlib/Elements/Three-Phase Parallel RLC Load  LConnTagsString=A|B|C  Configuration=Y (grounded)  NominalVoltage=(33000)*0.880402  Vabc=[1e3 1e3 1e3]  Vabcp=[1e3 1e3 1e3]  NominalFrequency=60  UnbalancedPower=off  ActivePower=11.2e6  InductivePower=7.5e6  CapacitivePower=0  Pabc=[10e3 9e3 11e3]  QLabc=[100 90 110]  QCabc=[100 90 110]  Pabcp=[10e3 9e3 11e3]  QLabcp=[100 90 110]  QCabcp=[100 90 110]  Measurements=None  LoadType=constant PQ
  Load14 : powerlib/Elements/Three-Phase Parallel RLC Load  LConnTagsString=A|B|C  Configuration=Y (grounded)  NominalVoltage=(33000)*0.859866  Vabc=[1e3 1e3 1e3]  Vabcp=[1e3 1e3 1e3]  NominalFrequency=60  UnbalancedPower=off  ActivePower=6.2e6  InductivePower=1.6e6  CapacitivePower=0  Pabc=[10e3 9e3 11e3]  QLabc=[100 90 110]  QCabc=[100 90 110]  Pabcp=[10e3 9e3 11e3]  QLabcp=[100 90 110]  QCabcp=[100 90 110]  Measurements=None  LoadType=constant PQ
  Load15 : powerlib/Elements/Three-Phase Parallel RLC Load  LConnTagsString=A|B|C  Configuration=Y (grounded)  NominalVoltage=(33000)*0.851164  Vabc=[1e3 1e3 1e3]  Vabcp=[1e3 1e3 1e3]  NominalFrequency=60  UnbalancedPower=off  ActivePower=8.2e6  InductivePower=2.5e6  CapacitivePower=0  Pabc=[10e3 9e3 11e3]  QLabc=[100 90 110]  QCabc=[100 90 110]  Pabcp=[10e3 9e3 11e3]  QLabcp=[100 90 110]  QCabcp=[100 90 110]  Measurements=None  LoadType=constant PQ
  Load16 : powerlib/Elements/Three-Phase Parallel RLC Load  LConnTagsString=A|B|C  Configuration=Y (grounded)  NominalVoltage=(33000)*0.850987  Vabc=[1e3 1e3 1e3]  Vabcp=[1e3 1e3 1e3]  NominalFrequency=60  UnbalancedPower=off  ActivePower=3.5e6  InductivePower=1.8e6  CapacitivePower=0  Pabc=[10e3 9e3 11e3]  QLabc=[100 90 110]  QCabc=[100 90 110]  Pabcp=[10e3 9e3 11e3]  QLabcp=[100 90 110]  QCabcp=[100 90 110]  Measurements=None  LoadType=constant PQ
  Load17 : powerlib/Elements/Three-Phase Parallel RLC Load  LConnTagsString=A|B|C  Configuration=Y (grounded)  NominalVoltage=(33000)*0.834792  Vabc=[1e3 1e3 1e3]  Vabcp=[1e3 1e3 1e3]  NominalFrequency=60  UnbalancedPower=off  ActivePower=9e6  InductivePower=5.8e6  CapacitivePower=0  Pabc=[10e3 9e3 11e3]  QLabc=[100 90 110]  QCabc=[100 90 110]  Pabcp=[10e3 9e3 11e3]  QLabcp=[100 90 110]  QCabcp=[100 90 110]  Measurements=None  LoadType=constant PQ
  Load18 : powerlib/Elements/Three-Phase Parallel RLC Load  LConnTagsString=A|B|C  Configuration=Y (grounded)  NominalVoltage=(33000)*0.830582  Vabc=[1e3 1e3 1e3]  Vabcp=[1e3 1e3 1e3]  NominalFrequency=60  UnbalancedPower=off  ActivePower=3.2e6  InductivePower=0.9e6  CapacitivePower=0  Pabc=[10e3 9e3 11e3]  QLabc=[100 90 110]  QCabc=[100 90 110]  Pabcp=[10e3 9e3 11e3]  QLabcp=[100 90 110]  QCabcp=[100 90 110]  Measurements=None  LoadType=constant PQ
  Load19 : powerlib/Elements/Three-Phase Parallel RLC Load  LConnTagsString=A|B|C  Configuration=Y (grounded)  NominalVoltage=(33000)*0.822392  Vabc=[1e3 1e3 1e3]  Vabcp=[1e3 1e3 1e3]  NominalFrequency=60  UnbalancedPower=off  ActivePower=9.5e6  InductivePower=3.4e6  CapacitivePower=0  Pabc=[10e3 9e3 11e3]  QLabc=[100 90 110]  QCabc=[100 90 110]  Pabcp=[10e3 9e3 11e3]  QLabcp=[100 90 110]  QCabcp=[100 90 110]  Measurements=None  LoadType=constant PQ
  Load2 : powerlib/Elements/Three-Phase Parallel RLC Load  LConnTagsString=A|B|C  Configuration=Y (grounded)  NominalVoltage=(132000)*1.01913  Vabc=[1e3 1e3 1e3]  Vabcp=[1e3 1e3 1e3]  NominalFrequency=60  UnbalancedPower=off  ActivePower=21.7e6  InductivePower=12.7e6  CapacitivePower=0  Pabc=[10e3 9e3 11e3]  QLabc=[100 90 110]  QCabc=[100 90 110]  Pabcp=[10e3 9e3 11e3]  QLabcp=[100 90 110]  QCabcp=[100 90 110]  Measurements=None  LoadType=constant PQ
  Load20 : powerlib/Elements/Three-Phase Parallel RLC Load  LConnTagsString=A|B|C  Configuration=Y (grounded)  NominalVoltage=(33000)*0.824807  Vabc=[1e3 1e3 1e3]  Vabcp=[1e3 1e3 1e3]  NominalFrequency=60  UnbalancedPower=off  ActivePower=2.2e6  InductivePower=0.7e6  CapacitivePower=0  Pabc=[10e3 9e3 11e3]  QLabc=[100 90 110]  QCabc=[100 90 110]  Pabcp=[10e3 9e3 11e3]  QLabcp=[100 90 110]  QCabcp=[100 90 110]  Measurements=None  LoadType=constant PQ
  Load21 : powerlib/Elements/Three-Phase Parallel RLC Load  LConnTagsString=A|B|C  Configuration=Y (grounded)  NominalVoltage=(33000)*0.821699  Vabc=[1e3 1e3 1e3]  Vabcp=[1e3 1e3 1e3]  NominalFrequency=60  UnbalancedPower=off  ActivePower=17.5e6  InductivePower=11.2e6  CapacitivePower=0  Pabc=[10e3 9e3 11e3]  QLabc=[100 90 110]  QCabc=[100 90 110]  Pabcp=[10e3 9e3 11e3]  QLabcp=[100 90 110]  QCabcp=[100 90 110]  Measurements=None  LoadType=constant PQ
  Load23 : powerlib/Elements/Three-Phase Parallel RLC Load  LConnTagsString=A|B|C  Configuration=Y (grounded)  NominalVoltage=(33000)*0.836572  Vabc=[1e3 1e3 1e3]  Vabcp=[1e3 1e3 1e3]  NominalFrequency=60  UnbalancedPower=off  ActivePower=3.2e6  InductivePower=1.6e6  CapacitivePower=0  Pabc=[10e3 9e3 11e3]  QLabc=[100 90 110]  QCabc=[100 90 110]  Pabcp=[10e3 9e3 11e3]  QLabcp=[100 90 110]  QCabcp=[100 90 110]  Measurements=None  LoadType=constant PQ
  Load24 : powerlib/Elements/Three-Phase Parallel RLC Load  LConnTagsString=A|B|C  Configuration=Y (grounded)  NominalVoltage=(33000)*0.827428  Vabc=[1e3 1e3 1e3]  Vabcp=[1e3 1e3 1e3]  NominalFrequency=60  UnbalancedPower=off  ActivePower=8.7e6  InductivePower=6.7e6  CapacitivePower=0  Pabc=[10e3 9e3 11e3]  QLabc=[100 90 110]  QCabc=[100 90 110]  Pabcp=[10e3 9e3 11e3]  QLabcp=[100 90 110]  QCabcp=[100 90 110]  Measurements=None  LoadType=constant PQ
  Load26 : powerlib/Elements/Three-Phase Parallel RLC Load  LConnTagsString=A|B|C  Configuration=Y (grounded)  NominalVoltage=(33000)*0.839219  Vabc=[1e3 1e3 1e3]  Vabcp=[1e3 1e3 1e3]  NominalFrequency=60  UnbalancedPower=off  ActivePower=3.5e6  InductivePower=2.3e6  CapacitivePower=0  Pabc=[10e3 9e3 11e3]  QLabc=[100 90 110]  QCabc=[100 90 110]  Pabcp=[10e3 9e3 11e3]  QLabcp=[100 90 110]  QCabcp=[100 90 110]  Measurements=None  LoadType=constant PQ
  Load29 : powerlib/Elements/Three-Phase Parallel RLC Load  LConnTagsString=A|B|C  Configuration=Y (grounded)  NominalVoltage=(33000)*0.867619  Vabc=[1e3 1e3 1e3]  Vabcp=[1e3 1e3 1e3]  NominalFrequency=60  UnbalancedPower=off  ActivePower=2.4e6  InductivePower=0.9e6  CapacitivePower=0  Pabc=[10e3 9e3 11e3]  QLabc=[100 90 110]  QCabc=[100 90 110]  Pabcp=[10e3 9e3 11e3]  QLabcp=[100 90 110]  QCabcp=[100 90 110]  Measurements=None  LoadType=constant PQ
  Load3 : powerlib/Elements/Three-Phase Parallel RLC Load  LConnTagsString=A|B|C  Configuration=Y (grounded)  NominalVoltage=(132000)*0.979973  Vabc=[1e3 1e3 1e3]  Vabcp=[1e3 1e3 1e3]  NominalFrequency=60  UnbalancedPower=off  ActivePower=2.4e6  InductivePower=1.2e6  CapacitivePower=0  Pabc=[10e3 9e3 11e3]  QLabc=[100 90 110]  QCabc=[100 90 110]  Pabcp=[10e3 9e3 11e3]  QLabcp=[100 90 110]  QCabcp=[100 90 110]  Measurements=None  LoadType=constant PQ
  Load30 : powerlib/Elements/Three-Phase Parallel RLC Load  LConnTagsString=A|B|C  Configuration=Y (grounded)  NominalVoltage=(33000)*0.854228  Vabc=[1e3 1e3 1e3]  Vabcp=[1e3 1e3 1e3]  NominalFrequency=60  UnbalancedPower=off  ActivePower=10.6e6  InductivePower=1.9e6  CapacitivePower=0  Pabc=[10e3 9e3 11e3]  QLabc=[100 90 110]  QCabc=[100 90 110]  Pabcp=[10e3 9e3 11e3]  QLabcp=[100 90 110]  QCabcp=[100 90 110]  Measurements=None  LoadType=constant PQ
  Load4 : powerlib/Elements/Three-Phase Parallel RLC Load  LConnTagsString=A|B|C  Configuration=Y (grounded)  NominalVoltage=(132000)*0.961405  Vabc=[1e3 1e3 1e3]  Vabcp=[1e3 1e3 1e3]  NominalFrequency=60  UnbalancedPower=off  ActivePower=7.6e6  InductivePower=1.6e6  CapacitivePower=0  Pabc=[10e3 9e3 11e3]  QLabc=[100 90 110]  QCabc=[100 90 110]  Pabcp=[10e3 9e3 11e3]  QLabcp=[100 90 110]  QCabcp=[100 90 110]  Measurements=None  LoadType=constant PQ
  Load5 : powerlib/Elements/Three-Phase Parallel RLC Load  LConnTagsString=A|B|C  Configuration=Y (grounded)  NominalVoltage=(132000)*0.970336  Vabc=[1e3 1e3 1e3]  Vabcp=[1e3 1e3 1e3]  NominalFrequency=60  UnbalancedPower=off  ActivePower=94.2e6  InductivePower=19e6  CapacitivePower=0  Pabc=[10e3 9e3 11e3]  QLabc=[100 90 110]  QCabc=[100 90 110]  Pabcp=[10e3 9e3 11e3]  QLabcp=[100 90 110]  QCabcp=[100 90 110]  Measurements=None  LoadType=constant PQ
  Load7 : powerlib/Elements/Three-Phase Parallel RLC Load  LConnTagsString=A|B|C  Configuration=Y (grounded)  NominalVoltage=(132000)*0.952342  Vabc=[1e3 1e3 1e3]  Vabcp=[1e3 1e3 1e3]  NominalFrequency=60  UnbalancedPower=off  ActivePower=22.8e6  InductivePower=10.9e6  CapacitivePower=0  Pabc=[10e3 9e3 11e3]  QLabc=[100 90 110]  QCabc=[100 90 110]  Pabcp=[10e3 9e3 11e3]  QLabcp=[100 90 110]  QCabcp=[100 90 110]  Measurements=None  LoadType=constant PQ
  Load8 : powerlib/Elements/Three-Phase Parallel RLC Load  LConnTagsString=A|B|C  Configuration=Y (grounded)  NominalVoltage=(132000)*0.953629  Vabc=[1e3 1e3 1e3]  Vabcp=[1e3 1e3 1e3]  NominalFrequency=60  UnbalancedPower=off  ActivePower=30e6  InductivePower=30e6  CapacitivePower=0  Pabc=[10e3 9e3 11e3]  QLabc=[100 90 110]  QCabc=[100 90 110]  Pabcp=[10e3 9e3 11e3]  QLabcp=[100 90 110]  QCabcp=[100 90 110]  Measurements=None  LoadType=constant PQ
  T1 : powerlib/Elements/Three-Phase Transformer (Two Windings)  Winding1Connection=Yg  Winding2Connection=Yg  CoreType=Three single-phase transformers  SetSaturation=off  Hysteresis=off  DataFile='hysteresis'  SetInitialFlux=off  Measurements=None  UNITS=pu  NominalPower=[ 100e6 , 60 ]  Winding1=[132e3 1e-6 0]  Winding2=[33e3 1e-6 0.256]  Rm=500  Lm=500  L0=0.5  Saturation=[0 0;8.6418e-06 0.00075383;0.0036007 0.00095485]  InitialFluxes=[0.00050255 -0.00050255 0.00043973]  MoreParameters=off  BreakLoop=off  DataType=off  TransfoNumber=1
  T2 : powerlib/Elements/Three-Phase Transformer (Two Windings)  Winding1Connection=Yg  Winding2Connection=Yg  CoreType=Three single-phase transformers  SetSaturation=off  Hysteresis=off  DataFile='hysteresis'  SetInitialFlux=off  Measurements=None  UNITS=pu  NominalPower=[ 100e6 , 60 ]  Winding1=[132e3 1e-6 0]  Winding2=[33e3 1e-6 0.556]  Rm=500  Lm=500  L0=0.5  Saturation=[0 0;8.6418e-06 0.00075383;0.0036007 0.00095485]  InitialFluxes=[0.00050255 -0.00050255 0.00043973]  MoreParameters=off  BreakLoop=off  DataType=off  TransfoNumber=1
  T3 : powerlib/Elements/Three-Phase Transformer (Two Windings)  Winding1Connection=Yg  Winding2Connection=Yg  CoreType=Three single-phase transformers  SetSaturation=off  Hysteresis=off  DataFile='hysteresis'  SetInitialFlux=off  Measurements=None  UNITS=pu  NominalPower=[ 100e6 , 60 ]  Winding1=[132e3 1e-6 0]  Winding2=[33e3 1e-6 0.208]  Rm=500  Lm=500  L0=0.5  Saturation=[0 0;8.6418e-06 0.00075383;0.0036007 0.00095485]  InitialFluxes=[0.00050255 -0.00050255 0.00043973]  MoreParameters=off  BreakLoop=off  DataType=off  TransfoNumber=1
  T3_12-13 : powerlib/Elements/Three-Phase Series RLC Branch  LConnTagsString=A|B|C  RConnTagsString=A|B|C  BranchType=L  Resistance=0  Inductance=0.14  Capacitance=1e-6  Measurements=None
  T3_9-10 : powerlib/Elements/Three-Phase Series RLC Branch  LConnTagsString=A|B|C  RConnTagsString=A|B|C  BranchType=L  Resistance=0  Inductance=0.11  Capacitance=1e-6  Measurements=None
  T3_9-11 : powerlib/Elements/Three-Phase Series RLC Branch  LConnTagsString=A|B|C  RConnTagsString=A|B|C  BranchType=L  Resistance=0  Inductance=0.208  Capacitance=1e-6  Measurements=None
  T4 : powerlib/Elements/Three-Phase Transformer (Two Windings)  Winding1Connection=Yg  Winding2Connection=Yg  CoreType=Three single-phase transformers  SetSaturation=off  Hysteresis=off  DataFile='hysteresis'  SetInitialFlux=off  Measurements=None  UNITS=pu  NominalPower=[ 100e6 , 60 ]  Winding1=[132e3 1e-6 0]  Winding2=[33e3 1e-6 0.396]  Rm=500  Lm=500  L0=0.5  Saturation=[0 0;8.6418e-06 0.00075383;0.0036007 0.00095485]  InitialFluxes=[0.00050255 -0.00050255 0.00043973]  MoreParameters=off  BreakLoop=off  DataType=off  TransfoNumber=1
  powergui : powerlib/powergui  Priority=1  SimulationMode=Phasor  SampleTime=50e-6  frequency=60  Iterations=50  frequencyindice=60  Pbase=100E6  ErrMax=1e-05  UnitsV=kV  UnitsW=MW  buscounter=0  FunctionMessages=off  echomessages=off  EnableUseOfTLC=off  CurrentSourceSwitches=off  DisableSnubberDevices=off  DisableRonSwitches=off  DisableVfSwitches=off  DisplayEquations=off  SolverType=Tustin/Backward Euler (TBE)  Interpol=off  ExternalGateDelay=off  methode=off  Ts=100  x0status=blocks  SPID=on  SwTol=0  HookPort=off  RestoreLinks=warning  ResistiveCurrentMeasurement=off  Frange=[0:2:500]  Ylog=off  Xlog=on  ShowGrid=off  save=off  variable=ZData  structure=0  ZoomFFT=off  StartTime=0.0  cycles=1  DisplayStyle=1  fundamental=60  FreqAxis=off  MaxFrequency=1000  frequencyindicesteady=1  RmsSteady=1  display=off
  connections:
  Bus2/RConn5 -- G2/RConn2
  G2/RConn3 -- Bus2/RConn6
  G2/RConn1 -- Bus2/RConn4
  Load2/LConn1 -- Bus2/RConn1
  Load2/LConn2 -- Bus2/RConn2
  Load2/LConn3 -- Bus2/RConn3
  Bus3/LConn6 -- Load3/LConn3
  Load3/LConn2 -- Bus3/LConn5
  Load3/LConn1 -- Bus3/LConn4
  Line 1-2-1/LConn2 -- Bus1/RConn5
  Line 1-2-1/LConn1 -- Bus1/RConn6
  Line 1-2-1/LConn3 -- Bus1/RConn4
  Line 1-2-2/LConn1 -- Line 1-2-1/RConn1 -- Fault 1-2/LConn1
  Line 1-2-2/LConn2 -- Line 1-2-1/RConn2 -- Fault 1-2/LConn2
  Line 1-2-2/LConn3 -- Line 1-2-1/RConn3 -- Fault 1-2/LConn3
  Line 1-2-2/RConn1 -- Bus2/LConn1
  Line 1-2-2/RConn2 -- Bus2/LConn2
  Line 1-2-2/RConn3 -- Bus2/LConn3
  Line 1-3-1/LConn2 -- Bus1/RConn2
  Line 1-3-1/LConn1 -- Bus1/RConn1 -- Load Flow Bus7/LConn1
  Line 1-3-1/LConn3 -- Bus1/RConn3
  Line 1-3-2/RConn2 -- Bus3/LConn2
  Bus3/LConn1 -- Line 1-3-2/RConn1
  Bus3/LConn3 -- Line 1-3-2/RConn3
  Line 3-4-1/LConn2 -- Bus3/RConn2
  Line 3-4-2/RConn2 -- Bus4/LConn2
  Line 3-4-2/RConn1 -- Load Flow Bus3/LConn1 -- Bus4/LConn1
  Line 3-4-2/RConn3 -- Bus4/LConn3
  Line 3-4-2/LConn1 -- Fault 3-4/LConn1 -- Line 3-4-1/RConn1
  Line 3-4-2/LConn2 -- Fault 3-4/LConn2 -- Line 3-4-1/RConn2
  Line 3-4-2/LConn3 -- Fault 3-4/LConn3 -- Line 3-4-1/RConn3
  Line 2-4-2/RConn2 -- Bus4/LConn5
  Line 2-4-2/RConn1 -- Bus4/LConn4
  Line 2-4-2/RConn3 -- Bus4/LConn6
  Line 2-4-2/LConn1 -- Line 2-4-1/RConn1 -- Fault 2-4/LConn1
  Line 2-4-1/RConn2 -- Fault 2-4/LConn2 -- Line 2-4-2/LConn2
  Line 2-4-2/LConn3 -- Line 2-4-1/RConn3 -- Fault 2-4/LConn3
  Bus2/LConn5 -- Line 2-4-1/LConn2
  Line 2-4-1/LConn1 -- Bus2/LConn4
  Line 2-4-1/LConn3 -- Bus2/LConn6
  Line 2-5-1/LConn1 -- Bus2/RConn7
  Bus2/RConn8 -- Line 2-5-1/LConn2
  Bus2/RConn9 -- Line 2-5-1/LConn3
  Line 2-5-1/RConn1 -- Fault 2-5/LConn1 -- Line 2-5-2/LConn1
  Line 2-5-1/RConn2 -- Fault 2-5/LConn2 -- Line 2-5-2/LConn2
  Line 2-5-1/RConn3 -- Fault 2-5/LConn3 -- Line 2-5-2/LConn3
  Line 2-5-2/RConn1 -- Bus5/LConn1 -- Load Flow Bus4/LConn1
  Line 2-5-2/RConn2 -- Bus5/LConn2
  Line 2-5-2/RConn3 -- Bus5/LConn3
  Line 2-6-1/LConn3 -- Load Flow Bus1/LConn1 -- Bus2/LConn9
  Line 2-6-1/LConn2 -- Bus2/LConn8
  Line 2-6-1/LConn1 -- Bus2/LConn7
  Line 2-6-1/RConn1 -- Fault 2-6/LConn1 -- Line 2-6-2/LConn1
  Line 2-6-1/RConn2 -- Fault 2-6/LConn2 -- Line 2-6-2/LConn2
  Line 2-6-1/RConn3 -- Fault 2-6/LConn3 -- Line 2-6-2/LConn3
  Bus6/LConn1 -- Line 2-6-2/RConn1
  Bus6/LConn2 -- Line 2-6-2/RConn2
  Line 2-6-2/RConn3 -- Bus6/LConn3
  G5/RConn1 -- Bus5/RConn1
  G5/RConn2 -- Bus5/RConn2
  G5/RConn3 -- Bus5/RConn3
  Load5/LConn2 -- Bus5/RConn5
  Load5/LConn3 -- Bus5/RConn6
  Load5/LConn1 -- Bus5/RConn4
  Line 3-4-1/LConn3 -- Bus3/RConn3
  Line 3-4-1/LConn1 -- Load Flow Bus2/LConn1 -- Bus3/RConn1
  Bus5/LConn4 -- Line 5-7-1/LConn1
  Line 5-7-1/LConn2 -- Bus5/LConn5
  Bus5/LConn6 -- Line 5-7-1/LConn3
  Line 5-7-2/LConn1 -- Fault 5-7/LConn1 -- Line 5-7-1/RConn1
  Line 5-7-2/LConn2 -- Fault 5-7/LConn2 -- Line 5-7-1/RConn2
  Line 5-7-2/LConn3 -- Fault 5-7/LConn3 -- Line 5-7-1/RConn3
  Bus7/LConn4 -- Line 5-7-2/RConn1
  Bus7/LConn5 -- Line 5-7-2/RConn2
  Bus7/LConn6 -- Line 5-7-2/RConn3
  Load7/LConn1 -- Load Flow Bus6/LConn1 -- Bus7/LConn1
  Load7/LConn2 -- Bus7/LConn2
  Load7/LConn3 -- Bus7/LConn3
  Line 6-7-1/LConn2 -- Bus6/LConn5
  Line 6-7-1/LConn3 -- Bus6/LConn6
  Line 6-7-1/LConn1 -- Bus6/LConn4
  Line 6-7-2/RConn1 -- Bus7/LConn7
  Line 6-7-2/RConn2 -- Bus7/LConn8
  Line 6-7-2/RConn3 -- Bus7/LConn9
  Fault 6-7/LConn1 -- Line 6-7-2/LConn1 -- Line 6-7-1/RConn1
  Fault 6-7/LConn2 -- Line 6-7-2/LConn2 -- Line 6-7-1/RConn2
  Fault 6-7/LConn3 -- Line 6-7-2/LConn3 -- Line 6-7-1/RConn3
  Line 6-8-1/LConn2 -- Bus6/LConn8
  Line 6-8-1/LConn1 -- Bus6/LConn7
  Line 6-8-1/LConn3 -- Bus6/LConn9
  Fault 6-8/LConn1 -- Line 6-8-1/RConn1 -- Line 6-8-2/LConn1
  Line 6-8-2/LConn2 -- Line 6-8-1/RConn2 -- Fault 6-8/LConn2
  Line 6-8-2/LConn3 -- Line 6-8-1/RConn3 -- Fault 6-8/LConn3
  Bus8/LConn3 -- Line 6-8-2/RConn3
  Bus8/LConn2 -- Line 6-8-2/RConn2
  Bus8/LConn1 -- Line 6-8-2/RConn1 -- Load Flow Bus8/LConn1
  Load8/LConn1 -- Bus8/RConn4
  Bus8/RConn5 -- Load8/LConn2
  Load8/LConn3 -- Bus8/RConn6
  Line 4-6-1/LConn2 -- Bus4/LConn8
  Line 4-6-1/LConn1 -- Bus4/LConn7
  Line 4-6-1/LConn3 -- Bus4/LConn9
  Line 4-6-2/RConn2 -- Bus6/RConn2
  Line 4-6-2/RConn1 -- Bus6/RConn1
  Line 4-6-2/RConn3 -- Bus6/RConn3
  Fault 4-6/LConn1 -- Line 4-6-2/LConn1 -- Line 4-6-1/RConn1
  Fault 4-6/LConn2 -- Line 4-6-2/LConn2 -- Line 4-6-1/RConn2
  Fault 4-6/LConn3 -- Line 4-6-2/LConn3 -- Line 4-6-1/RConn3
  T2/RConn2 -- Bus10/LConn2
  T2/RConn1 -- Load Flow Bus10/LConn1 -- Bus10/LConn1
  T2/RConn3 -- Bus10/LConn3
  T2/LConn1 -- Bus6/RConn4
  T2/LConn2 -- Bus6/RConn5
  T2/LConn3 -- Bus6/RConn6
  T3/RConn2 -- Bus9/LConn2
  T3/RConn1 -- Load Flow Bus9/LConn1 -- Bus9/LConn1
  T3/RConn3 -- Bus9/LConn3
  T3/LConn1 -- Bus6/RConn7
  T3/LConn2 -- Bus6/RConn8
  T3/LConn3 -- Bus6/RConn9
  T3_9-10/RConn2 -- Bus10/LConn5
  Bus9/RConn1 -- T3_9-10/LConn1
  Bus9/RConn2 -- T3_9-10/LConn2
  Bus9/RConn3 -- T3_9-10/LConn3
  T3_9-10/RConn1 -- Bus10/LConn4
  T3_9-10/RConn3 -- Bus10/LConn6
  Load10/LConn1 -- Bus10/LConn7
  Load10/LConn2 -- Bus10/LConn8
  Load10/LConn3 -- Bus10/LConn9
  G11/RConn1 -- Load Flow Bus11/LConn1 -- Bus11/RConn1
  G11/RConn2 -- Bus11/RConn2
  G11/RConn3 -- Bus11/RConn3
  Bus9/RConn6 -- T3_9-11/LConn3
  Bus9/RConn5 -- T3_9-11/LConn2
  T3_9-11/LConn1 -- Bus9/RConn4
  Bus11/LConn1 -- T3_9-11/RConn1
  Bus11/LConn2 -- T3_9-11/RConn2
  Bus11/LConn3 -- T3_9-11/RConn3
  T1/LConn2 -- Bus4/RConn2
  T1/LConn1 -- Bus4/RConn1
  T1/LConn3 -- Bus4/RConn3
  Bus12/LConn8 -- T1/RConn2
  T1/RConn3 -- Bus12/LConn9
  T1/RConn1 -- Bus12/LConn7
  T3_12-13/RConn1 -- Bus12/LConn4
  T3_12-13/RConn2 -- Bus12/LConn5
  T3_12-13/RConn3 -- Bus12/LConn6
  Bus13/LConn1 -- Load Flow Bus13/LConn1 -- T3_12-13/LConn1
  Bus13/LConn2 -- T3_12-13/LConn2
  Bus13/LConn3 -- T3_12-13/LConn3
  G13/RConn1 -- Bus13/RConn1
  G13/RConn2 -- Bus13/RConn2
  G13/RConn3 -- Bus13/RConn3
  Line 12-14-1/LConn2 -- Bus12/RConn2
  Line 12-14-1/LConn1 -- Bus12/RConn1
  Line 12-14-1/LConn3 -- Bus12/RConn3
  Fault 12-14/LConn3 -- Line 12-14-1/RConn3 -- Line 12-14-2/LConn3
  Fault 12-14/LConn2 -- Line 12-14-2/LConn2 -- Line 12-14-1/RConn2
  Fault 12-14/LConn1 -- Line 12-14-2/LConn1 -- Line 12-14-1/RConn1
  Load14/LConn1 -- Bus14/LConn1
  Bus14/LConn2 -- Load14/LConn2
  Load14/LConn3 -- Bus14/LConn3
  Line 14-15-1/LConn3 -- Bus14/RConn3
  Line 14-15-1/LConn2 -- Bus14/RConn2
  Line 14-15-1/LConn1 -- Load Flow Bus14/LConn1 -- Bus14/RConn1
  Line 14-15-2/LConn1 -- Fault 14-15/LConn1 -- Line 14-15-1/RConn1
  Line 14-15-2/LConn2 -- Fault 14-15/LConn2 -- Line 14-15-1/RConn2
  Line 14-15-2/LConn3 -- Fault 14-15/LConn3 -- Line 14-15-1/RConn3
  Line 14-15-2/RConn1 -- Load Flow Bus15/LConn1 -- Bus15/LConn1
  Line 14-15-2/RConn2 -- Bus15/LConn2
  Line 14-15-2/RConn3 -- Bus15/LConn3
  Line 12-15-2/RConn1 -- Bus15/LConn4
  Line 12-15-2/RConn2 -- Bus15/LConn5
  Line 12-15-2/RConn3 -- Bus15/LConn6
  Line 12-15-2/LConn1 -- Line 12-15-1/RConn1 -- Fault 12-15/LConn1
  Line 12-15-2/LConn2 -- Line 12-15-1/RConn2 -- Fault 12-15/LConn2
  Line 12-15-2/LConn3 -- Line 12-15-1/RConn3 -- Fault 12-15/LConn3
  Load15/LConn1 -- Bus15/RConn1
  Bus15/RConn2 -- Load15/LConn2
  Load15/LConn3 -- Bus15/RConn3
  Line 15-18-2/RConn2 -- Bus18/LConn2
  Line 15-18-2/RConn1 -- Bus18/LConn1
  Line 15-18-2/RConn3 -- Bus18/LConn3
  Line 15-18-1/RConn1 -- Fault 15-18/LConn1 -- Line 15-18-2/LConn1
  Line 15-18-2/LConn2 -- Fault 15-18/LConn2 -- Line 15-18-1/RConn2
  Line 15-18-1/RConn3 -- Fault 15-18/LConn3 -- Line 15-18-2/LConn3
  Line 15-18-1/LConn1 -- Bus15/LConn7
  Line 15-18-1/LConn2 -- Bus15/LConn8
  Line 15-18-1/LConn3 -- Bus15/LConn9
  Bus18/RConn2 -- Load18/LConn2
  Load18/LConn1 -- Load Flow Bus18/LConn1 -- Bus18/RConn1
  Load18/LConn3 -- Bus18/RConn3
  Line 18-19-1/RConn2 -- Bus18/LConn5
  Line 18-19-1/RConn1 -- Bus18/LConn4
  Line 18-19-1/RConn3 -- Bus18/LConn6
  Line 18-19-1/LConn1 -- Fault 18-19/LConn1 -- Line 18-19-2/LConn1
  Line 18-19-2/LConn2 -- Fault 18-19/LConn2 -- Line 18-19-1/LConn2
  Line 18-19-1/LConn3 -- Fault 18-19/LConn3 -- Line 18-19-2/LConn3
  Line 18-19-2/RConn1 -- Bus19/LConn1
  Bus19/LConn2 -- Line 18-19-2/RConn2
  Line 18-19-2/RConn3 -- Bus19/LConn3
  Bus19/RConn2 -- Load19/LConn2
  Load19/LConn1 -- Load Flow Bus19/LConn1 -- Bus19/RConn1
  Load19/LConn3 -- Bus19/RConn3
  Fault 12-16/LConn3 -- Line 12-16-1/RConn3 -- Line 12-16-2/LConn3
  Fault 12-16/LConn2 -- Line 12-16-1/RConn2 -- Line 12-16-2/LConn2
  Line 12-16-2/LConn1 -- Line 12-16-1/RConn1 -- Fault 12-16/LConn1
  Line 12-16-2/RConn1 -- Bus16/LConn1 -- Load Flow Bus16/LConn1
  Line 12-16-2/RConn2 -- Bus16/LConn2
  Line 12-16-2/RConn3 -- Bus16/LConn3
  Line 10-17-1/LConn2 -- Bus10/RConn2
  Line 10-17-1/LConn1 -- Bus10/RConn1
  Line 10-17-1/LConn3 -- Bus10/RConn3
  Line 10-17-2/LConn1 -- Line 10-17-1/RConn1 -- Fault 10-17/LConn1
  Line 10-17-2/LConn3 -- Fault 10-17/LConn3 -- Line 10-17-1/RConn3
  Line 10-17-2/LConn2 -- Fault 10-17/LConn2 -- Line 10-17-1/RConn2
  Line 10-17-2/RConn2 -- Bus17/LConn5
  Line 10-17-2/RConn3 -- Bus17/LConn6
  Line 10-17-2/RConn1 -- Bus17/LConn4
  Line 16-17-1/LConn1 -- Bus16/LConn4
  Bus16/LConn5 -- Line 16-17-1/LConn2
  Line 16-17-1/LConn3 -- Bus16/LConn6
  Line 16-17-2/LConn1 -- Fault 16-17/LConn1 -- Line 16-17-1/RConn1
  Line 16-17-2/LConn2 -- Fault 16-17/LConn2 -- Line 16-17-1/RConn2
  Line 16-17-2/LConn3 -- Fault 16-17/LConn3 -- Line 16-17-1/RConn3
  Line 16-17-2/RConn1 -- Bus17/LConn1
  Line 16-17-2/RConn2 -- Bus17/LConn2
  Line 16-17-2/RConn3 -- Bus17/LConn3
  Load17/LConn2 -- Bus17/RConn2
  Load17/LConn1 -- Load Flow Bus17/LConn1 -- Bus17/RConn1
  Load17/LConn3 -- Bus17/RConn3
  Line 19-20-2/RConn2 -- Bus20/LConn2
  Line 19-20-2/RConn1 -- Bus20/LConn1
  Line 19-20-2/RConn3 -- Bus20/LConn3
  Line 19-20-1/LConn2 -- Bus19/LConn5
  Line 19-20-1/RConn2 -- Fault 19-20/LConn2 -- Line 19-20-2/LConn2
  Line 19-20-1/RConn1 -- Fault 19-20/LConn1 -- Line 19-20-2/LConn1
  Fault 19-20/LConn3 -- Line 19-20-1/RConn3 -- Line 19-20-2/LConn3
  Line 10-20-2/RConn2 -- Bus20/LConn5
  Line 10-20-2/RConn1 -- Bus20/LConn4
  Line 10-20-2/RConn3 -- Bus20/LConn6
  Line 10-20-1/RConn1 -- Line 10-20-2/LConn1 -- Fault 10-20/LConn1
  Line 10-20-1/RConn2 -- Line 10-20-2/LConn2 -- Fault 10-20/LConn2
  Line 10-20-1/RConn3 -- Line 10-20-2/LConn3 -- Fault 10-20/LConn3
  Line 10-20-1/LConn1 -- Bus10/RConn4
  Line 10-20-1/LConn2 -- Bus10/RConn5
  Line 10-20-1/LConn3 -- Bus10/RConn6
  Load20/LConn2 -- Bus20/RConn2
  Load20/LConn1 -- Load Flow Bus20/LConn1 -- Bus20/RConn1
  Load20/LConn3 -- Bus20/RConn3
  Load21/LConn2 -- Bus21/RConn2
  Load21/LConn1 -- Load Flow Bus21/LConn1 -- Bus21/RConn1
  Load21/LConn3 -- Bus21/RConn3
  Line 10-21-2/RConn2 -- Bus21/LConn2
  Line 10-21-2/RConn1 -- Bus21/LConn1
  Line 10-21-2/RConn3 -- Bus21/LConn3
  Line 10-21-1/RConn1 -- Line 10-21-2/LConn1 -- Fault 10-21/LConn1
  Line 10-21-1/RConn2 -- Line 10-21-2/LConn2 -- Fault 10-21/LConn2
  Line 10-21-1/RConn3 -- Line 10-21-2/LConn3 -- Fault 10-21/LConn3
  Line 10-21-1/LConn1 -- Bus10/RConn7
  Line 10-21-1/LConn2 -- Bus10/RConn8
  Line 10-21-1/LConn3 -- Bus10/RConn9
  Line 21-22-2/RConn2 -- Bus22/LConn2
  Line 21-22-2/RConn3 -- Bus22/LConn3
  Line 21-22-2/RConn1 -- Bus22/LConn1
  Line 21-22-1/RConn2 -- Bus21/LConn5
  Line 21-22-1/RConn3 -- Bus21/LConn6
  Line 21-22-1/RConn1 -- Bus21/LConn4
  Line 21-22-1/LConn3 -- Fault 21-22/LConn3 -- Line 21-22-2/LConn3
  Line 21-22-1/LConn2 -- Fault 21-22/LConn2 -- Line 21-22-2/LConn2
  Line 21-22-1/LConn1 -- Fault 21-22/LConn1 -- Line 21-22-2/LConn1
  Line 10-22-2/RConn2 -- Bus22/LConn5
  Line 10-22-2/RConn3 -- Bus22/LConn6
  Line 10-22-2/RConn1 -- Bus22/LConn4
  Line 10-22-1/RConn1 -- Line 10-22-2/LConn1 -- Fault 10-22/LConn1
  Line 10-22-1/RConn2 -- Line 10-22-2/LConn2 -- Fault 10-22/LConn2
  Line 10-22-1/RConn3 -- Line 10-22-2/LConn3 -- Fault 10-22/LConn3
  Line 10-22-1/LConn1 -- Bus10/RConn10
  Line 10-22-1/LConn2 -- Bus10/RConn11
  Bus10/RConn12 -- Line 10-22-1/LConn3
  Load23/LConn2 -- Bus23/RConn2
  Load23/LConn1 -- Load Flow Bus23/LConn1 -- Bus23/RConn1
  Load23/LConn3 -- Bus23/RConn3
  Line 15-23-1/LConn2 -- Bus15/RConn5
  Line 15-23-1/LConn1 -- Bus15/RConn4
  Line 15-23-1/LConn3 -- Bus15/RConn6
  Line 15-23-2/RConn1 -- Bus23/LConn1
  Line 15-23-2/RConn2 -- Bus23/LConn2
  Line 15-23-2/RConn3 -- Bus23/LConn3
  Line 15-23-2/LConn3 -- Fault 15-23/LConn3 -- Line 15-23-1/RConn3
  Line 15-23-2/LConn2 -- Fault 15-23/LConn2 -- Line 15-23-1/RConn2
  Line 15-23-2/LConn1 -- Fault 15-23/LConn1 -- Line 15-23-1/RConn1
  Line 23-24-1/LConn1 -- Bus23/LConn4
  Line 23-24-1/LConn2 -- Bus23/LConn5
  Line 23-24-1/LConn3 -- Bus23/LConn6
  Line 23-24-2/LConn1 -- Fault 23-24/LConn1 -- Line 23-24-1/RConn1
  Line 23-24-2/LConn2 -- Fault 23-24/LConn2 -- Line 23-24-1/RConn2
  Line 23-24-2/LConn3 -- Fault 23-24/LConn3 -- Line 23-24-1/RConn3
  Line 23-24-2/RConn1 -- Bus24/LConn1 -- Load Flow Bus24/LConn1
  Line 23-24-2/RConn2 -- Bus24/LConn2
  Line 23-24-2/RConn3 -- Bus24/LConn3
  Line 22-24-1/LConn2 -- Bus22/RConn2
  Line 22-24-1/LConn1 -- Load Flow Bus22/LConn1 -- Bus22/RConn1
  Line 22-24-1/LConn3 -- Bus22/RConn3
  Line 22-24-2/RConn1 -- Bus24/LConn4
  Bus24/LConn5 -- Line 22-24-2/RConn2
  Line 22-24-2/RConn3 -- Bus24/LConn6
  Line 22-24-2/LConn1 -- Fault 22-24/LConn1 -- Line 22-24-1/RConn1
  Line 22-24-2/LConn2 -- Fault 22-24/LConn2 -- Line 22-24-1/RConn2
  Line 22-24-2/LConn3 -- Fault 22-24/LConn3 -- Line 22-24-1/RConn3
  Load24/LConn1 -- Bus24/RConn1
  Load24/LConn2 -- Bus24/RConn2
  Load24/LConn3 -- Bus24/RConn3
  Line 24-25-1/LConn2 -- Bus24/RConn5
  Line 24-25-1/LConn1 -- Bus24/RConn4
  Line 24-25-1/LConn3 -- Bus24/RConn6
  Line 24-25-2/RConn1 -- Bus25/LConn1 -- Load Flow Bus25/LConn1
  Line 24-25-2/RConn2 -- Bus25/LConn2
  Line 24-25-2/RConn3 -- Bus25/LConn3
  Line 24-25-1/RConn3 -- Fault 24-25/LConn3 -- Line 24-25-2/LConn3
  Line 24-25-1/RConn2 -- Fault 24-25/LConn2 -- Line 24-25-2/LConn2
  Line 24-25-1/RConn1 -- Fault 24-25/LConn1 -- Line 24-25-2/LConn1
  G8/RConn1 -- Bus8/RConn7
  G8/RConn2 -- Bus8/RConn8
  G8/RConn3 -- Bus8/RConn9
  Line 25-26-1/LConn2 -- Bus25/LConn5
  Line 25-26-1/LConn1 -- Bus25/LConn4
  Line 25-26-1/LConn3 -- Bus25/LConn6
  Line 25-26-2/RConn1 -- Bus26/LConn1
  Line 25-26-2/RConn2 -- Bus26/LConn2
  Line 25-26-2/RConn3 -- Bus26/LConn3
  Line 25-26-2/LConn1 -- Fault 25-26/LConn1 -- Line 25-26-1/RConn1
  Line 25-26-2/LConn2 -- Fault 25-26/LConn2 -- Line 25-26-1/RConn2
  Line 25-26-1/RConn3 -- Fault 25-26/LConn3 -- Line 25-26-2/LConn3
  Load26/LConn2 -- Bus26/RConn2
  Load26/LConn1 -- Load Flow Bus26/LConn1 -- Bus26/RConn1
  Bus26/RConn3 -- Load26/LConn3
  Line 25-27-1/RConn2 -- Bus25/RConn2
  Line 25-27-1/RConn1 -- Bus25/RConn1
  Line 25-27-1/RConn3 -- Bus25/RConn3
  Line 25-27-2/LConn3 -- Fault 25-27/LConn3 -- Line 25-27-1/LConn3
  Line 25-27-2/LConn2 -- Fault 25-27/LConn2 -- Line 25-27-1/LConn2
  Line 25-27-2/LConn1 -- Fault 25-27/LConn1 -- Line 25-27-1/LConn1
  Line 25-27-2/RConn1 -- Bus27/LConn7 -- Load Flow Bus27/LConn1
  Bus27/LConn8 -- Line 25-27-2/RConn2
  Bus27/LConn9 -- Line 25-27-2/RConn3
  Line 27-30-1/LConn1 -- Bus27/LConn4
  Line 27-30-1/LConn2 -- Bus27/LConn5
  Line 27-30-1/LConn3 -- Bus27/LConn6
  Line 27-30-2/LConn1 -- Fault 27-30/LConn1 -- Line 27-30-1/RConn1
  Line 27-30-2/LConn2 -- Fault 27-30/LConn2 -- Line 27-30-1/RConn2
  Line 27-30-2/LConn3 -- Fault 27-30/LConn3 -- Line 27-30-1/RConn3
  Bus30/RConn5 -- Line 27-30-2/RConn2
  Line 27-30-2/RConn1 -- Bus30/RConn4
  Line 27-30-2/RConn3 -- Bus30/RConn6
  Load30/LConn2 -- Bus30/LConn2
  Load30/LConn1 -- Load Flow Bus30/LConn1 -- Bus30/LConn1
  Load30/LConn3 -- Bus30/LConn3
  Line 29-30-2/LConn1 -- Bus30/RConn1
  Line 29-30-2/LConn2 -- Bus30/RConn2
  Line 29-30-2/LConn3 -- Bus30/RConn3
  Line 29-30-1/RConn1 -- Fault 29-30/LConn1 -- Line 29-30-2/RConn1
  Line 29-30-2/RConn2 -- Fault 29-30/LConn2 -- Line 29-30-1/RConn2
  Line 29-30-2/RConn3 -- Fault 29-30/LConn3 -- Line 29-30-1/RConn3
  Line 29-30-1/LConn2 -- Bus29/RConn2
  Line 29-30-1/LConn1 -- Bus29/RConn1
  Line 29-30-1/LConn3 -- Bus29/RConn3
  Line 27-29-2/RConn2 -- Bus29/RConn5
  Line 27-29-2/RConn1 -- Bus29/RConn4
  Line 27-29-2/RConn3 -- Bus29/RConn6
  Line 27-29-1/LConn1 -- Bus27/LConn1
  Line 27-29-1/LConn2 -- Bus27/LConn2
  Line 27-29-1/LConn3 -- Bus27/LConn3
  Fault 27-29/LConn3 -- Line 27-29-2/LConn1 -- Line 27-29-1/RConn1
  Fault 27-29/LConn2 -- Line 27-29-2/LConn2 -- Line 27-29-1/RConn2
  Fault 27-29/LConn1 -- Line 27-29-2/LConn3 -- Line 27-29-1/RConn3
  Load29/LConn2 -- Bus29/LConn2
  Load29/LConn1 -- Load Flow Bus29/LConn1 -- Bus29/LConn1
  Bus29/LConn3 -- Load29/LConn3
  T4/RConn1 -- Bus27/RConn1
  T4/RConn2 -- Bus27/RConn2
  T4/RConn3 -- Bus27/RConn3
  T4/LConn1 -- Load Flow Bus28/LConn1 -- Bus28/LConn1
  T4/LConn2 -- Bus28/LConn2
  T4/LConn3 -- Bus28/LConn3
  Line 8-28-1/LConn3 -- Bus8/RConn3
  Line 8-28-1/LConn2 -- Bus8/RConn2
  Line 8-28-1/LConn1 -- Bus8/RConn1
  Line 8-28-2/LConn1 -- Fault 8-28/LConn1 -- Line 8-28-1/RConn1
  Line 8-28-2/LConn2 -- Fault 8-28/LConn2 -- Line 8-28-1/RConn2
  Line 8-28-2/LConn3 -- Fault 8-28/LConn3 -- Line 8-28-1/RConn3
  Bus28/RConn3 -- Line 8-28-2/RConn1
  Line 8-28-2/RConn2 -- Bus28/RConn2
  Bus28/RConn1 -- Line 8-28-2/RConn3
  Line 6-28-1/LConn1 -- Load Flow Bus5/LConn1 -- Bus6/RConn10
  Bus6/RConn11 -- Line 6-28-1/LConn2
  Line 6-28-1/LConn3 -- Bus6/RConn12
  Line 6-28-2/LConn1 -- Fault 6-28/LConn1 -- Line 6-28-1/RConn1
  Line 6-28-2/LConn2 -- Fault 6-28/LConn2 -- Line 6-28-1/RConn2
  Line 6-28-2/LConn3 -- Fault 6-28/LConn3 -- Line 6-28-1/RConn3
  Bus28/RConn6 -- Line 6-28-2/RConn1
  Bus28/RConn5 -- Line 6-28-2/RConn2
  Line 6-28-2/RConn3 -- Bus28/RConn4
  G1/RConn2 -- Bus1/LConn2
  G1/RConn1 -- Bus1/LConn1
  G1/RConn3 -- Bus1/LConn3
  Line 12-16-1/LConn2 -- Bus12/RConn8
  Line 12-16-1/LConn3 -- Bus12/RConn9
  Line 12-16-1/LConn1 -- Bus12/RConn7
  Line 12-15-1/LConn2 -- Bus12/RConn5
  Line 12-15-1/LConn1 -- Bus12/RConn4
  Line 12-15-1/LConn3 -- Bus12/RConn6
  Line 12-14-2/RConn2 -- Bus14/LConn5
  Line 12-14-2/RConn1 -- Bus14/LConn4
  Line 12-14-2/RConn3 -- Bus14/LConn6
  Load16/LConn2 -- Bus16/RConn2
  Load16/LConn1 -- Bus16/RConn1
  Load16/LConn3 -- Bus16/RConn3
  Line 19-20-1/LConn3 -- Bus19/LConn6
  Line 19-20-1/LConn1 -- Bus19/LConn4
  Line 1-3-1/RConn1 -- Line 1-3-2/LConn1 -- Fault 1-3/LConn1
  Line 1-3-1/RConn2 -- Line 1-3-2/LConn2 -- Fault 1-3/LConn2
  Line 1-3-1/RConn3 -- Line 1-3-2/LConn3 -- Fault 1-3/LConn3
  Load4/LConn2 -- Bus4/RConn5
  Load4/LConn1 -- Bus4/RConn4
  Load4/LConn3 -- Bus4/RConn6
  Load12/LConn1 -- Load Flow Bus12/LConn1 -- Bus12/LConn1
  Load12/LConn2 -- Bus12/LConn2
  Load12/LConn3 -- Bus12/LConn3
